simulink library "MBDS_Subsystems"  (R2018b)
settings: Solver=ode45  StartTime=0.0  StopTime=10.0  RelTol=1e-3
undefined symbols (not defined in the file or in its folder): nbo_False, nbo_True
libraries: KIBES_Signal x1438, MBDS_Modules x44, simulink x2
(part 11 of 15)

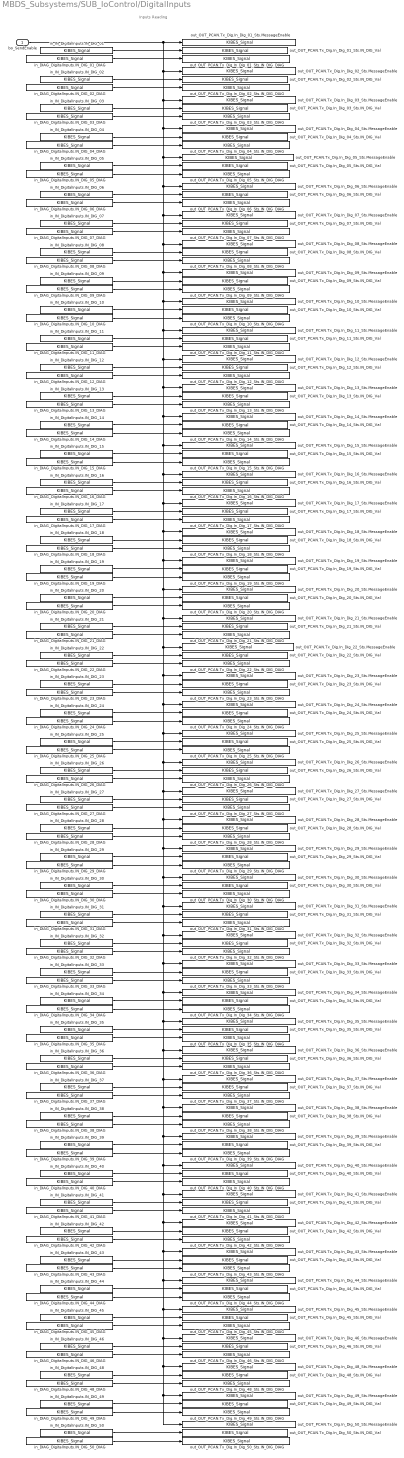
== system MBDS_Subsystems/SUB_IoControl/DigitalInputs ==
  note: Inputs Reading
  bo_SendEnable : Inport
  in_DIAG_DigitalInputs.IN_DIG_01_DIAG : KIBES_Signal/KIBES_Signal  MBDS_LibraryBlock=on  DatabaseKey=5  SignalName=DIAG_DigitalInputs.IN_DIG_01_DIAG  SymbolName=DIAG_DigitalInputs_IN_DIG_01_DIAG_000005  DataType=uint16  Init=1  Slope=1  Bias=0  DataSize=1  fpDataType=uint16  BlockIOType=Inport  DeviceType=0
  in_DIAG_DigitalInputs.IN_DIG_02_DIAG : KIBES_Signal/KIBES_Signal  MBDS_LibraryBlock=on  DatabaseKey=36  SignalName=DIAG_DigitalInputs.IN_DIG_02_DIAG  SymbolName=DIAG_DigitalInputs_IN_DIG_02_DIAG_000036  DataType=uint16  Init=1  Slope=1  Bias=0  DataSize=1  fpDataType=uint16  BlockIOType=Inport  DeviceType=0
  in_DIAG_DigitalInputs.IN_DIG_03_DIAG : KIBES_Signal/KIBES_Signal  MBDS_LibraryBlock=on  DatabaseKey=38  SignalName=DIAG_DigitalInputs.IN_DIG_03_DIAG  SymbolName=DIAG_DigitalInputs_IN_DIG_03_DIAG_000038  DataType=uint16  Init=1  Slope=1  Bias=0  DataSize=1  fpDataType=uint16  BlockIOType=Inport  DeviceType=0
  in_DIAG_DigitalInputs.IN_DIG_04_DIAG : KIBES_Signal/KIBES_Signal  MBDS_LibraryBlock=on  DatabaseKey=40  SignalName=DIAG_DigitalInputs.IN_DIG_04_DIAG  SymbolName=DIAG_DigitalInputs_IN_DIG_04_DIAG_000040  DataType=uint16  Init=1  Slope=1  Bias=0  DataSize=1  fpDataType=uint16  BlockIOType=Inport  DeviceType=0
  in_DIAG_DigitalInputs.IN_DIG_05_DIAG : KIBES_Signal/KIBES_Signal  MBDS_LibraryBlock=on  DatabaseKey=88  SignalName=DIAG_DigitalInputs.IN_DIG_05_DIAG  SymbolName=DIAG_DigitalInputs_IN_DIG_05_DIAG_000088  DataType=uint16  Init=1  Slope=1  Bias=0  DataSize=1  fpDataType=uint16  BlockIOType=Inport  DeviceType=0
  in_DIAG_DigitalInputs.IN_DIG_06_DIAG : KIBES_Signal/KIBES_Signal  MBDS_LibraryBlock=on  DatabaseKey=93  SignalName=DIAG_DigitalInputs.IN_DIG_06_DIAG  SymbolName=DIAG_DigitalInputs_IN_DIG_06_DIAG_000093  DataType=uint16  Init=1  Slope=1  Bias=0  DataSize=1  fpDataType=uint16  BlockIOType=Inport  DeviceType=0
  in_DIAG_DigitalInputs.IN_DIG_07_DIAG : KIBES_Signal/KIBES_Signal  MBDS_LibraryBlock=on  DatabaseKey=89  SignalName=DIAG_DigitalInputs.IN_DIG_07_DIAG  SymbolName=DIAG_DigitalInputs_IN_DIG_07_DIAG_000089  DataType=uint16  Init=1  Slope=1  Bias=0  DataSize=1  fpDataType=uint16  BlockIOType=Inport  DeviceType=0
  in_DIAG_DigitalInputs.IN_DIG_08_DIAG : KIBES_Signal/KIBES_Signal  MBDS_LibraryBlock=on  DatabaseKey=90  SignalName=DIAG_DigitalInputs.IN_DIG_08_DIAG  SymbolName=DIAG_DigitalInputs_IN_DIG_08_DIAG_000090  DataType=uint16  Init=1  Slope=1  Bias=0  DataSize=1  fpDataType=uint16  BlockIOType=Inport  DeviceType=0
  in_DIAG_DigitalInputs.IN_DIG_09_DIAG : KIBES_Signal/KIBES_Signal  MBDS_LibraryBlock=on  DatabaseKey=95  SignalName=DIAG_DigitalInputs.IN_DIG_09_DIAG  SymbolName=DIAG_DigitalInputs_IN_DIG_09_DIAG_000095  DataType=uint16  Init=1  Slope=1  Bias=0  DataSize=1  fpDataType=uint16  BlockIOType=Inport  DeviceType=0
  in_DIAG_DigitalInputs.IN_DIG_10_DIAG : KIBES_Signal/KIBES_Signal  MBDS_LibraryBlock=on  DatabaseKey=97  SignalName=DIAG_DigitalInputs.IN_DIG_10_DIAG  SymbolName=DIAG_DigitalInputs_IN_DIG_10_DIAG_000097  DataType=uint16  Init=1  Slope=1  Bias=0  DataSize=1  fpDataType=uint16  BlockIOType=Inport  DeviceType=0
  in_DIAG_DigitalInputs.IN_DIG_11_DIAG : KIBES_Signal/KIBES_Signal  MBDS_LibraryBlock=on  DatabaseKey=99  SignalName=DIAG_DigitalInputs.IN_DIG_11_DIAG  SymbolName=DIAG_DigitalInputs_IN_DIG_11_DIAG_000099  DataType=uint16  Init=1  Slope=1  Bias=0  DataSize=1  fpDataType=uint16  BlockIOType=Inport  DeviceType=0
  in_DIAG_DigitalInputs.IN_DIG_12_DIAG : KIBES_Signal/KIBES_Signal  MBDS_LibraryBlock=on  DatabaseKey=101  SignalName=DIAG_DigitalInputs.IN_DIG_12_DIAG  SymbolName=DIAG_DigitalInputs_IN_DIG_12_DIAG_000101  DataType=uint16  Init=1  Slope=1  Bias=0  DataSize=1  fpDataType=uint16  BlockIOType=Inport  DeviceType=0
  in_DIAG_DigitalInputs.IN_DIG_13_DIAG : KIBES_Signal/KIBES_Signal  MBDS_LibraryBlock=on  DatabaseKey=9  SignalName=DIAG_DigitalInputs.IN_DIG_13_DIAG  SymbolName=DIAG_DigitalInputs_IN_DIG_13_DIAG_000009  DataType=uint16  Init=1  Slope=1  Bias=0  DataSize=1  fpDataType=uint16  BlockIOType=Inport  DeviceType=0
  in_DIAG_DigitalInputs.IN_DIG_14_DIAG : KIBES_Signal/KIBES_Signal  MBDS_LibraryBlock=on  DatabaseKey=11  SignalName=DIAG_DigitalInputs.IN_DIG_14_DIAG  SymbolName=DIAG_DigitalInputs_IN_DIG_14_DIAG_000011  DataType=uint16  Init=1  Slope=1  Bias=0  DataSize=1  fpDataType=uint16  BlockIOType=Inport  DeviceType=0
  in_DIAG_DigitalInputs.IN_DIG_15_DIAG : KIBES_Signal/KIBES_Signal  MBDS_LibraryBlock=on  DatabaseKey=13  SignalName=DIAG_DigitalInputs.IN_DIG_15_DIAG  SymbolName=DIAG_DigitalInputs_IN_DIG_15_DIAG_000013  DataType=uint16  Init=1  Slope=1  Bias=0  DataSize=1  fpDataType=uint16  BlockIOType=Inport  DeviceType=0
  in_DIAG_DigitalInputs.IN_DIG_16_DIAG : KIBES_Signal/KIBES_Signal  MBDS_LibraryBlock=on  DatabaseKey=15  SignalName=DIAG_DigitalInputs.IN_DIG_16_DIAG  SymbolName=DIAG_DigitalInputs_IN_DIG_16_DIAG_000015  DataType=uint16  Init=1  Slope=1  Bias=0  DataSize=1  fpDataType=uint16  BlockIOType=Inport  DeviceType=0
  in_DIAG_DigitalInputs.IN_DIG_17_DIAG : KIBES_Signal/KIBES_Signal  MBDS_LibraryBlock=on  DatabaseKey=17  SignalName=DIAG_DigitalInputs.IN_DIG_17_DIAG  SymbolName=DIAG_DigitalInputs_IN_DIG_17_DIAG_000017  DataType=uint16  Init=1  Slope=1  Bias=0  DataSize=1  fpDataType=uint16  BlockIOType=Inport  DeviceType=0
  in_DIAG_DigitalInputs.IN_DIG_18_DIAG : KIBES_Signal/KIBES_Signal  MBDS_LibraryBlock=on  DatabaseKey=19  SignalName=DIAG_DigitalInputs.IN_DIG_18_DIAG  SymbolName=DIAG_DigitalInputs_IN_DIG_18_DIAG_000019  DataType=uint16  Init=1  Slope=1  Bias=0  DataSize=1  fpDataType=uint16  BlockIOType=Inport  DeviceType=0
  in_DIAG_DigitalInputs.IN_DIG_19_DIAG : KIBES_Signal/KIBES_Signal  MBDS_LibraryBlock=on  DatabaseKey=21  SignalName=DIAG_DigitalInputs.IN_DIG_19_DIAG  SymbolName=DIAG_DigitalInputs_IN_DIG_19_DIAG_000021  DataType=uint16  Init=1  Slope=1  Bias=0  DataSize=1  fpDataType=uint16  BlockIOType=Inport  DeviceType=0
  in_DIAG_DigitalInputs.IN_DIG_20_DIAG : KIBES_Signal/KIBES_Signal  MBDS_LibraryBlock=on  DatabaseKey=23  SignalName=DIAG_DigitalInputs.IN_DIG_20_DIAG  SymbolName=DIAG_DigitalInputs_IN_DIG_20_DIAG_000023  DataType=uint16  Init=1  Slope=1  Bias=0  DataSize=1  fpDataType=uint16  BlockIOType=Inport  DeviceType=0
  in_DIAG_DigitalInputs.IN_DIG_21_DIAG : KIBES_Signal/KIBES_Signal  MBDS_LibraryBlock=on  DatabaseKey=25  SignalName=DIAG_DigitalInputs.IN_DIG_21_DIAG  SymbolName=DIAG_DigitalInputs_IN_DIG_21_DIAG_000025  DataType=uint16  Init=1  Slope=1  Bias=0  DataSize=1  fpDataType=uint16  BlockIOType=Inport  DeviceType=0
  in_DIAG_DigitalInputs.IN_DIG_22_DIAG : KIBES_Signal/KIBES_Signal  MBDS_LibraryBlock=on  DatabaseKey=27  SignalName=DIAG_DigitalInputs.IN_DIG_22_DIAG  SymbolName=DIAG_DigitalInputs_IN_DIG_22_DIAG_000027  DataType=uint16  Init=1  Slope=1  Bias=0  DataSize=1  fpDataType=uint16  BlockIOType=Inport  DeviceType=0
  in_DIAG_DigitalInputs.IN_DIG_23_DIAG : KIBES_Signal/KIBES_Signal  MBDS_LibraryBlock=on  DatabaseKey=29  SignalName=DIAG_DigitalInputs.IN_DIG_23_DIAG  SymbolName=DIAG_DigitalInputs_IN_DIG_23_DIAG_000029  DataType=uint16  Init=1  Slope=1  Bias=0  DataSize=1  fpDataType=uint16  BlockIOType=Inport  DeviceType=0
  in_DIAG_DigitalInputs.IN_DIG_24_DIAG : KIBES_Signal/KIBES_Signal  MBDS_LibraryBlock=on  DatabaseKey=31  SignalName=DIAG_DigitalInputs.IN_DIG_24_DIAG  SymbolName=DIAG_DigitalInputs_IN_DIG_24_DIAG_000031  DataType=uint16  Init=1  Slope=1  Bias=0  DataSize=1  fpDataType=uint16  BlockIOType=Inport  DeviceType=0
  in_DIAG_DigitalInputs.IN_DIG_25_DIAG : KIBES_Signal/KIBES_Signal  MBDS_LibraryBlock=on  DatabaseKey=33  SignalName=DIAG_DigitalInputs.IN_DIG_25_DIAG  SymbolName=DIAG_DigitalInputs_IN_DIG_25_DIAG_000033  DataType=uint16  Init=1  Slope=1  Bias=0  DataSize=1  fpDataType=uint16  BlockIOType=Inport  DeviceType=0
  in_DIAG_DigitalInputs.IN_DIG_26_DIAG : KIBES_Signal/KIBES_Signal  MBDS_LibraryBlock=on  DatabaseKey=41  SignalName=DIAG_DigitalInputs.IN_DIG_26_DIAG  SymbolName=DIAG_DigitalInputs_IN_DIG_26_DIAG_000041  DataType=uint16  Init=1  Slope=1  Bias=0  DataSize=1  fpDataType=uint16  BlockIOType=Inport  DeviceType=0
  in_DIAG_DigitalInputs.IN_DIG_27_DIAG : KIBES_Signal/KIBES_Signal  MBDS_LibraryBlock=on  DatabaseKey=43  SignalName=DIAG_DigitalInputs.IN_DIG_27_DIAG  SymbolName=DIAG_DigitalInputs_IN_DIG_27_DIAG_000043  DataType=uint16  Init=1  Slope=1  Bias=0  DataSize=1  fpDataType=uint16  BlockIOType=Inport  DeviceType=0
  in_DIAG_DigitalInputs.IN_DIG_28_DIAG : KIBES_Signal/KIBES_Signal  MBDS_LibraryBlock=on  DatabaseKey=45  SignalName=DIAG_DigitalInputs.IN_DIG_28_DIAG  SymbolName=DIAG_DigitalInputs_IN_DIG_28_DIAG_000045  DataType=uint16  Init=1  Slope=1  Bias=0  DataSize=1  fpDataType=uint16  BlockIOType=Inport  DeviceType=0
  in_DIAG_DigitalInputs.IN_DIG_29_DIAG : KIBES_Signal/KIBES_Signal  MBDS_LibraryBlock=on  DatabaseKey=47  SignalName=DIAG_DigitalInputs.IN_DIG_29_DIAG  SymbolName=DIAG_DigitalInputs_IN_DIG_29_DIAG_000047  DataType=uint16  Init=1  Slope=1  Bias=0  DataSize=1  fpDataType=uint16  BlockIOType=Inport  DeviceType=0
  in_DIAG_DigitalInputs.IN_DIG_30_DIAG : KIBES_Signal/KIBES_Signal  MBDS_LibraryBlock=on  DatabaseKey=49  SignalName=DIAG_DigitalInputs.IN_DIG_30_DIAG  SymbolName=DIAG_DigitalInputs_IN_DIG_30_DIAG_000049  DataType=uint16  Init=1  Slope=1  Bias=0  DataSize=1  fpDataType=uint16  BlockIOType=Inport  DeviceType=0
  in_DIAG_DigitalInputs.IN_DIG_31_DIAG : KIBES_Signal/KIBES_Signal  MBDS_LibraryBlock=on  DatabaseKey=51  SignalName=DIAG_DigitalInputs.IN_DIG_31_DIAG  SymbolName=DIAG_DigitalInputs_IN_DIG_31_DIAG_000051  DataType=uint16  Init=1  Slope=1  Bias=0  DataSize=1  fpDataType=uint16  BlockIOType=Inport  DeviceType=0
  in_DIAG_DigitalInputs.IN_DIG_32_DIAG : KIBES_Signal/KIBES_Signal  MBDS_LibraryBlock=on  DatabaseKey=53  SignalName=DIAG_DigitalInputs.IN_DIG_32_DIAG  SymbolName=DIAG_DigitalInputs_IN_DIG_32_DIAG_000053  DataType=uint16  Init=1  Slope=1  Bias=0  DataSize=1  fpDataType=uint16  BlockIOType=Inport  DeviceType=0
  in_DIAG_DigitalInputs.IN_DIG_33_DIAG : KIBES_Signal/KIBES_Signal  MBDS_LibraryBlock=on  DatabaseKey=55  SignalName=DIAG_DigitalInputs.IN_DIG_33_DIAG  SymbolName=DIAG_DigitalInputs_IN_DIG_33_DIAG_000055  DataType=uint16  Init=1  Slope=1  Bias=0  DataSize=1  fpDataType=uint16  BlockIOType=Inport  DeviceType=0
  in_DIAG_DigitalInputs.IN_DIG_34_DIAG : KIBES_Signal/KIBES_Signal  MBDS_LibraryBlock=on  DatabaseKey=57  SignalName=DIAG_DigitalInputs.IN_DIG_34_DIAG  SymbolName=DIAG_DigitalInputs_IN_DIG_34_DIAG_000057  DataType=uint16  Init=1  Slope=1  Bias=0  DataSize=1  fpDataType=uint16  BlockIOType=Inport  DeviceType=0
  in_DIAG_DigitalInputs.IN_DIG_35_DIAG : KIBES_Signal/KIBES_Signal  MBDS_LibraryBlock=on  DatabaseKey=59  SignalName=DIAG_DigitalInputs.IN_DIG_35_DIAG  SymbolName=DIAG_DigitalInputs_IN_DIG_35_DIAG_000059  DataType=uint16  Init=1  Slope=1  Bias=0  DataSize=1  fpDataType=uint16  BlockIOType=Inport  DeviceType=0
  in_DIAG_DigitalInputs.IN_DIG_36_DIAG : KIBES_Signal/KIBES_Signal  MBDS_LibraryBlock=on  DatabaseKey=61  SignalName=DIAG_DigitalInputs.IN_DIG_36_DIAG  SymbolName=DIAG_DigitalInputs_IN_DIG_36_DIAG_000061  DataType=uint16  Init=1  Slope=1  Bias=0  DataSize=1  fpDataType=uint16  BlockIOType=Inport  DeviceType=0
  in_DIAG_DigitalInputs.IN_DIG_37_DIAG : KIBES_Signal/KIBES_Signal  MBDS_LibraryBlock=on  DatabaseKey=63  SignalName=DIAG_DigitalInputs.IN_DIG_37_DIAG  SymbolName=DIAG_DigitalInputs_IN_DIG_37_DIAG_000063  DataType=uint16  Init=1  Slope=1  Bias=0  DataSize=1  fpDataType=uint16  BlockIOType=Inport  DeviceType=0
  in_DIAG_DigitalInputs.IN_DIG_38_DIAG : KIBES_Signal/KIBES_Signal  MBDS_LibraryBlock=on  DatabaseKey=65  SignalName=DIAG_DigitalInputs.IN_DIG_38_DIAG  SymbolName=DIAG_DigitalInputs_IN_DIG_38_DIAG_000065  DataType=uint16  Init=1  Slope=1  Bias=0  DataSize=1  fpDataType=uint16  BlockIOType=Inport  DeviceType=0
  in_DIAG_DigitalInputs.IN_DIG_39_DIAG : KIBES_Signal/KIBES_Signal  MBDS_LibraryBlock=on  DatabaseKey=67  SignalName=DIAG_DigitalInputs.IN_DIG_39_DIAG  SymbolName=DIAG_DigitalInputs_IN_DIG_39_DIAG_000067  DataType=uint16  Init=1  Slope=1  Bias=0  DataSize=1  fpDataType=uint16  BlockIOType=Inport  DeviceType=0
  in_DIAG_DigitalInputs.IN_DIG_40_DIAG : KIBES_Signal/KIBES_Signal  MBDS_LibraryBlock=on  DatabaseKey=69  SignalName=DIAG_DigitalInputs.IN_DIG_40_DIAG  SymbolName=DIAG_DigitalInputs_IN_DIG_40_DIAG_000069  DataType=uint16  Init=1  Slope=1  Bias=0  DataSize=1  fpDataType=uint16  BlockIOType=Inport  DeviceType=0
  in_DIAG_DigitalInputs.IN_DIG_41_DIAG : KIBES_Signal/KIBES_Signal  MBDS_LibraryBlock=on  DatabaseKey=71  SignalName=DIAG_DigitalInputs.IN_DIG_41_DIAG  SymbolName=DIAG_DigitalInputs_IN_DIG_41_DIAG_000071  DataType=uint16  Init=1  Slope=1  Bias=0  DataSize=1  fpDataType=uint16  BlockIOType=Inport  DeviceType=0
  in_DIAG_DigitalInputs.IN_DIG_42_DIAG : KIBES_Signal/KIBES_Signal  MBDS_LibraryBlock=on  DatabaseKey=73  SignalName=DIAG_DigitalInputs.IN_DIG_42_DIAG  SymbolName=DIAG_DigitalInputs_IN_DIG_42_DIAG_000073  DataType=uint16  Init=1  Slope=1  Bias=0  DataSize=1  fpDataType=uint16  BlockIOType=Inport  DeviceType=0
  in_DIAG_DigitalInputs.IN_DIG_43_DIAG : KIBES_Signal/KIBES_Signal  MBDS_LibraryBlock=on  DatabaseKey=75  SignalName=DIAG_DigitalInputs.IN_DIG_43_DIAG  SymbolName=DIAG_DigitalInputs_IN_DIG_43_DIAG_000075  DataType=uint16  Init=1  Slope=1  Bias=0  DataSize=1  fpDataType=uint16  BlockIOType=Inport  DeviceType=0
  in_DIAG_DigitalInputs.IN_DIG_44_DIAG : KIBES_Signal/KIBES_Signal  MBDS_LibraryBlock=on  DatabaseKey=77  SignalName=DIAG_DigitalInputs.IN_DIG_44_DIAG  SymbolName=DIAG_DigitalInputs_IN_DIG_44_DIAG_000077  DataType=uint16  Init=1  Slope=1  Bias=0  DataSize=1  fpDataType=uint16  BlockIOType=Inport  DeviceType=0
  in_DIAG_DigitalInputs.IN_DIG_45_DIAG : KIBES_Signal/KIBES_Signal  MBDS_LibraryBlock=on  DatabaseKey=79  SignalName=DIAG_DigitalInputs.IN_DIG_45_DIAG  SymbolName=DIAG_DigitalInputs_IN_DIG_45_DIAG_000079  DataType=uint16  Init=1  Slope=1  Bias=0  DataSize=1  fpDataType=uint16  BlockIOType=Inport  DeviceType=0
  in_DIAG_DigitalInputs.IN_DIG_46_DIAG : KIBES_Signal/KIBES_Signal  MBDS_LibraryBlock=on  DatabaseKey=81  SignalName=DIAG_DigitalInputs.IN_DIG_46_DIAG  SymbolName=DIAG_DigitalInputs_IN_DIG_46_DIAG_000081  DataType=uint16  Init=1  Slope=1  Bias=0  DataSize=1  fpDataType=uint16  BlockIOType=Inport  DeviceType=0
  in_DIAG_DigitalInputs.IN_DIG_48_DIAG : KIBES_Signal/KIBES_Signal  MBDS_LibraryBlock=on  DatabaseKey=83  SignalName=DIAG_DigitalInputs.IN_DIG_48_DIAG  SymbolName=DIAG_DigitalInputs_IN_DIG_48_DIAG_000083  DataType=uint16  Init=1  Slope=1  Bias=0  DataSize=1  fpDataType=uint16  BlockIOType=Inport  DeviceType=0
  in_DIAG_DigitalInputs.IN_DIG_49_DIAG : KIBES_Signal/KIBES_Signal  MBDS_LibraryBlock=on  DatabaseKey=85  SignalName=DIAG_DigitalInputs.IN_DIG_49_DIAG  SymbolName=DIAG_DigitalInputs_IN_DIG_49_DIAG_000085  DataType=uint16  Init=1  Slope=1  Bias=0  DataSize=1  fpDataType=uint16  BlockIOType=Inport  DeviceType=0
  in_DIAG_DigitalInputs.IN_DIG_50_DIAG : KIBES_Signal/KIBES_Signal  MBDS_LibraryBlock=on  DatabaseKey=91  SignalName=DIAG_DigitalInputs.IN_DIG_50_DIAG  SymbolName=DIAG_DigitalInputs_IN_DIG_50_DIAG_000091  DataType=uint16  Init=1  Slope=1  Bias=0  DataSize=1  fpDataType=uint16  BlockIOType=Inport  DeviceType=0
  in_IN_DigitalInputs.IN_DIG_01 : KIBES_Signal/KIBES_Signal  MBDS_LibraryBlock=on  DatabaseKey=4  SignalName=IN_DigitalInputs.IN_DIG_01  SymbolName=IN_DigitalInputs_IN_DIG_01_000004  DataType=boolean  Init=0  Slope=1  Bias=0  DataSize=1  fpDataType=boolean  BlockIOType=Inport  DeviceType=0
  in_IN_DigitalInputs.IN_DIG_02 : KIBES_Signal/KIBES_Signal  MBDS_LibraryBlock=on  DatabaseKey=35  SignalName=IN_DigitalInputs.IN_DIG_02  SymbolName=IN_DigitalInputs_IN_DIG_02_000035  DataType=boolean  Init=0  Slope=1  Bias=0  DataSize=1  fpDataType=boolean  BlockIOType=Inport  DeviceType=0
  in_IN_DigitalInputs.IN_DIG_03 : KIBES_Signal/KIBES_Signal  MBDS_LibraryBlock=on  DatabaseKey=37  SignalName=IN_DigitalInputs.IN_DIG_03  SymbolName=IN_DigitalInputs_IN_DIG_03_000037  DataType=boolean  Init=0  Slope=1  Bias=0  DataSize=1  fpDataType=boolean  BlockIOType=Inport  DeviceType=0
  in_IN_DigitalInputs.IN_DIG_04 : KIBES_Signal/KIBES_Signal  MBDS_LibraryBlock=on  DatabaseKey=39  SignalName=IN_DigitalInputs.IN_DIG_04  SymbolName=IN_DigitalInputs_IN_DIG_04_000039  DataType=boolean  Init=0  Slope=1  Bias=0  DataSize=1  fpDataType=boolean  BlockIOType=Inport  DeviceType=0
  in_IN_DigitalInputs.IN_DIG_05 : KIBES_Signal/KIBES_Signal  MBDS_LibraryBlock=on  DatabaseKey=87  SignalName=IN_DigitalInputs.IN_DIG_05  SymbolName=IN_DigitalInputs_IN_DIG_05_000087  DataType=boolean  Init=0  Slope=1  Bias=0  DataSize=1  fpDataType=boolean  BlockIOType=Inport  DeviceType=0
  in_IN_DigitalInputs.IN_DIG_06 : KIBES_Signal/KIBES_Signal  MBDS_LibraryBlock=on  DatabaseKey=92  SignalName=IN_DigitalInputs.IN_DIG_06  SymbolName=IN_DigitalInputs_IN_DIG_06_000092  DataType=boolean  Init=0  Slope=1  Bias=0  DataSize=1  fpDataType=boolean  BlockIOType=Inport  DeviceType=0
  in_IN_DigitalInputs.IN_DIG_07 : KIBES_Signal/KIBES_Signal  MBDS_LibraryBlock=on  DatabaseKey=6  SignalName=IN_DigitalInputs.IN_DIG_07  SymbolName=IN_DigitalInputs_IN_DIG_07_000006  DataType=boolean  Init=0  Slope=1  Bias=0  DataSize=1  fpDataType=boolean  BlockIOType=Inport  DeviceType=0
  in_IN_DigitalInputs.IN_DIG_08 : KIBES_Signal/KIBES_Signal  MBDS_LibraryBlock=on  DatabaseKey=7  SignalName=IN_DigitalInputs.IN_DIG_08  SymbolName=IN_DigitalInputs_IN_DIG_08_000007  DataType=boolean  Init=0  Slope=1  Bias=0  DataSize=1  fpDataType=boolean  BlockIOType=Inport  DeviceType=0
  in_IN_DigitalInputs.IN_DIG_09 : KIBES_Signal/KIBES_Signal  MBDS_LibraryBlock=on  DatabaseKey=94  SignalName=IN_DigitalInputs.IN_DIG_09  SymbolName=IN_DigitalInputs_IN_DIG_09_000094  DataType=boolean  Init=0  Slope=1  Bias=0  DataSize=1  fpDataType=boolean  BlockIOType=Inport  DeviceType=0
  in_IN_DigitalInputs.IN_DIG_10 : KIBES_Signal/KIBES_Signal  MBDS_LibraryBlock=on  DatabaseKey=96  SignalName=IN_DigitalInputs.IN_DIG_10  SymbolName=IN_DigitalInputs_IN_DIG_10_000096  DataType=boolean  Init=0  Slope=1  Bias=0  DataSize=1  fpDataType=boolean  BlockIOType=Inport  DeviceType=0
  in_IN_DigitalInputs.IN_DIG_11 : KIBES_Signal/KIBES_Signal  MBDS_LibraryBlock=on  DatabaseKey=98  SignalName=IN_DigitalInputs.IN_DIG_11  SymbolName=IN_DigitalInputs_IN_DIG_11_000098  DataType=boolean  Init=0  Slope=1  Bias=0  DataSize=1  fpDataType=boolean  BlockIOType=Inport  DeviceType=0
  in_IN_DigitalInputs.IN_DIG_12 : KIBES_Signal/KIBES_Signal  MBDS_LibraryBlock=on  DatabaseKey=100  SignalName=IN_DigitalInputs.IN_DIG_12  SymbolName=IN_DigitalInputs_IN_DIG_12_000100  DataType=boolean  Init=0  Slope=1  Bias=0  DataSize=1  fpDataType=boolean  BlockIOType=Inport  DeviceType=0
  in_IN_DigitalInputs.IN_DIG_13 : KIBES_Signal/KIBES_Signal  MBDS_LibraryBlock=on  DatabaseKey=8  SignalName=IN_DigitalInputs.IN_DIG_13  SymbolName=IN_DigitalInputs_IN_DIG_13_000008  DataType=boolean  Init=0  Slope=1  Bias=0  DataSize=1  fpDataType=boolean  BlockIOType=Inport  DeviceType=0
  in_IN_DigitalInputs.IN_DIG_14 : KIBES_Signal/KIBES_Signal  MBDS_LibraryBlock=on  DatabaseKey=10  SignalName=IN_DigitalInputs.IN_DIG_14  SymbolName=IN_DigitalInputs_IN_DIG_14_000010  DataType=boolean  Init=0  Slope=1  Bias=0  DataSize=1  fpDataType=boolean  BlockIOType=Inport  DeviceType=0
  in_IN_DigitalInputs.IN_DIG_15 : KIBES_Signal/KIBES_Signal  MBDS_LibraryBlock=on  DatabaseKey=12  SignalName=IN_DigitalInputs.IN_DIG_15  SymbolName=IN_DigitalInputs_IN_DIG_15_000012  DataType=boolean  Init=0  Slope=1  Bias=0  DataSize=1  fpDataType=boolean  BlockIOType=Inport  DeviceType=0
  in_IN_DigitalInputs.IN_DIG_16 : KIBES_Signal/KIBES_Signal  MBDS_LibraryBlock=on  DatabaseKey=14  SignalName=IN_DigitalInputs.IN_DIG_16  SymbolName=IN_DigitalInputs_IN_DIG_16_000014  DataType=boolean  Init=0  Slope=1  Bias=0  DataSize=1  fpDataType=boolean  BlockIOType=Inport  DeviceType=0
  in_IN_DigitalInputs.IN_DIG_17 : KIBES_Signal/KIBES_Signal  MBDS_LibraryBlock=on  DatabaseKey=16  SignalName=IN_DigitalInputs.IN_DIG_17  SymbolName=IN_DigitalInputs_IN_DIG_17_000016  DataType=boolean  Init=0  Slope=1  Bias=0  DataSize=1  fpDataType=boolean  BlockIOType=Inport  DeviceType=0
  in_IN_DigitalInputs.IN_DIG_18 : KIBES_Signal/KIBES_Signal  MBDS_LibraryBlock=on  DatabaseKey=18  SignalName=IN_DigitalInputs.IN_DIG_18  SymbolName=IN_DigitalInputs_IN_DIG_18_000018  DataType=boolean  Init=0  Slope=1  Bias=0  DataSize=1  fpDataType=boolean  BlockIOType=Inport  DeviceType=0
  in_IN_DigitalInputs.IN_DIG_19 : KIBES_Signal/KIBES_Signal  MBDS_LibraryBlock=on  DatabaseKey=20  SignalName=IN_DigitalInputs.IN_DIG_19  SymbolName=IN_DigitalInputs_IN_DIG_19_000020  DataType=boolean  Init=0  Slope=1  Bias=0  DataSize=1  fpDataType=boolean  BlockIOType=Inport  DeviceType=0
  in_IN_DigitalInputs.IN_DIG_20 : KIBES_Signal/KIBES_Signal  MBDS_LibraryBlock=on  DatabaseKey=22  SignalName=IN_DigitalInputs.IN_DIG_20  SymbolName=IN_DigitalInputs_IN_DIG_20_000022  DataType=boolean  Init=0  Slope=1  Bias=0  DataSize=1  fpDataType=boolean  BlockIOType=Inport  DeviceType=0
  in_IN_DigitalInputs.IN_DIG_21 : KIBES_Signal/KIBES_Signal  MBDS_LibraryBlock=on  DatabaseKey=24  SignalName=IN_DigitalInputs.IN_DIG_21  SymbolName=IN_DigitalInputs_IN_DIG_21_000024  DataType=boolean  Init=0  Slope=1  Bias=0  DataSize=1  fpDataType=boolean  BlockIOType=Inport  DeviceType=0
  in_IN_DigitalInputs.IN_DIG_22 : KIBES_Signal/KIBES_Signal  MBDS_LibraryBlock=on  DatabaseKey=26  SignalName=IN_DigitalInputs.IN_DIG_22  SymbolName=IN_DigitalInputs_IN_DIG_22_000026  DataType=boolean  Init=0  Slope=1  Bias=0  DataSize=1  fpDataType=boolean  BlockIOType=Inport  DeviceType=0
  in_IN_DigitalInputs.IN_DIG_23 : KIBES_Signal/KIBES_Signal  MBDS_LibraryBlock=on  DatabaseKey=28  SignalName=IN_DigitalInputs.IN_DIG_23  SymbolName=IN_DigitalInputs_IN_DIG_23_000028  DataType=boolean  Init=0  Slope=1  Bias=0  DataSize=1  fpDataType=boolean  BlockIOType=Inport  DeviceType=0
  in_IN_DigitalInputs.IN_DIG_24 : KIBES_Signal/KIBES_Signal  MBDS_LibraryBlock=on  DatabaseKey=30  SignalName=IN_DigitalInputs.IN_DIG_24  SymbolName=IN_DigitalInputs_IN_DIG_24_000030  DataType=boolean  Init=0  Slope=1  Bias=0  DataSize=1  fpDataType=boolean  BlockIOType=Inport  DeviceType=0
  in_IN_DigitalInputs.IN_DIG_25 : KIBES_Signal/KIBES_Signal  MBDS_LibraryBlock=on  DatabaseKey=32  SignalName=IN_DigitalInputs.IN_DIG_25  SymbolName=IN_DigitalInputs_IN_DIG_25_000032  DataType=boolean  Init=0  Slope=1  Bias=0  DataSize=1  fpDataType=boolean  BlockIOType=Inport  DeviceType=0
  in_IN_DigitalInputs.IN_DIG_26 : KIBES_Signal/KIBES_Signal  MBDS_LibraryBlock=on  DatabaseKey=34  SignalName=IN_DigitalInputs.IN_DIG_26  SymbolName=IN_DigitalInputs_IN_DIG_26_000034  DataType=boolean  Init=0  Slope=1  Bias=0  DataSize=1  fpDataType=boolean  BlockIOType=Inport  DeviceType=0
  in_IN_DigitalInputs.IN_DIG_27 : KIBES_Signal/KIBES_Signal  MBDS_LibraryBlock=on  DatabaseKey=42  SignalName=IN_DigitalInputs.IN_DIG_27  SymbolName=IN_DigitalInputs_IN_DIG_27_000042  DataType=boolean  Init=0  Slope=1  Bias=0  DataSize=1  fpDataType=boolean  BlockIOType=Inport  DeviceType=0
  in_IN_DigitalInputs.IN_DIG_28 : KIBES_Signal/KIBES_Signal  MBDS_LibraryBlock=on  DatabaseKey=44  SignalName=IN_DigitalInputs.IN_DIG_28  SymbolName=IN_DigitalInputs_IN_DIG_28_000044  DataType=boolean  Init=0  Slope=1  Bias=0  DataSize=1  fpDataType=boolean  BlockIOType=Inport  DeviceType=0
  in_IN_DigitalInputs.IN_DIG_29 : KIBES_Signal/KIBES_Signal  MBDS_LibraryBlock=on  DatabaseKey=46  SignalName=IN_DigitalInputs.IN_DIG_29  SymbolName=IN_DigitalInputs_IN_DIG_29_000046  DataType=boolean  Init=0  Slope=1  Bias=0  DataSize=1  fpDataType=boolean  BlockIOType=Inport  DeviceType=0
  in_IN_DigitalInputs.IN_DIG_30 : KIBES_Signal/KIBES_Signal  MBDS_LibraryBlock=on  DatabaseKey=48  SignalName=IN_DigitalInputs.IN_DIG_30  SymbolName=IN_DigitalInputs_IN_DIG_30_000048  DataType=boolean  Init=0  Slope=1  Bias=0  DataSize=1  fpDataType=boolean  BlockIOType=Inport  DeviceType=0
  in_IN_DigitalInputs.IN_DIG_31 : KIBES_Signal/KIBES_Signal  MBDS_LibraryBlock=on  DatabaseKey=50  SignalName=IN_DigitalInputs.IN_DIG_31  SymbolName=IN_DigitalInputs_IN_DIG_31_000050  DataType=boolean  Init=0  Slope=1  Bias=0  DataSize=1  fpDataType=boolean  BlockIOType=Inport  DeviceType=0
  in_IN_DigitalInputs.IN_DIG_32 : KIBES_Signal/KIBES_Signal  MBDS_LibraryBlock=on  DatabaseKey=52  SignalName=IN_DigitalInputs.IN_DIG_32  SymbolName=IN_DigitalInputs_IN_DIG_32_000052  DataType=boolean  Init=0  Slope=1  Bias=0  DataSize=1  fpDataType=boolean  BlockIOType=Inport  DeviceType=0
  in_IN_DigitalInputs.IN_DIG_33 : KIBES_Signal/KIBES_Signal  MBDS_LibraryBlock=on  DatabaseKey=54  SignalName=IN_DigitalInputs.IN_DIG_33  SymbolName=IN_DigitalInputs_IN_DIG_33_000054  DataType=boolean  Init=0  Slope=1  Bias=0  DataSize=1  fpDataType=boolean  BlockIOType=Inport  DeviceType=0
  in_IN_DigitalInputs.IN_DIG_34 : KIBES_Signal/KIBES_Signal  MBDS_LibraryBlock=on  DatabaseKey=56  SignalName=IN_DigitalInputs.IN_DIG_34  SymbolName=IN_DigitalInputs_IN_DIG_34_000056  DataType=boolean  Init=0  Slope=1  Bias=0  DataSize=1  fpDataType=boolean  BlockIOType=Inport  DeviceType=0
  in_IN_DigitalInputs.IN_DIG_35 : KIBES_Signal/KIBES_Signal  MBDS_LibraryBlock=on  DatabaseKey=58  SignalName=IN_DigitalInputs.IN_DIG_35  SymbolName=IN_DigitalInputs_IN_DIG_35_000058  DataType=boolean  Init=0  Slope=1  Bias=0  DataSize=1  fpDataType=boolean  BlockIOType=Inport  DeviceType=0
  in_IN_DigitalInputs.IN_DIG_36 : KIBES_Signal/KIBES_Signal  MBDS_LibraryBlock=on  DatabaseKey=60  SignalName=IN_DigitalInputs.IN_DIG_36  SymbolName=IN_DigitalInputs_IN_DIG_36_000060  DataType=boolean  Init=0  Slope=1  Bias=0  DataSize=1  fpDataType=boolean  BlockIOType=Inport  DeviceType=0
  in_IN_DigitalInputs.IN_DIG_37 : KIBES_Signal/KIBES_Signal  MBDS_LibraryBlock=on  DatabaseKey=62  SignalName=IN_DigitalInputs.IN_DIG_37  SymbolName=IN_DigitalInputs_IN_DIG_37_000062  DataType=boolean  Init=0  Slope=1  Bias=0  DataSize=1  fpDataType=boolean  BlockIOType=Inport  DeviceType=0
  in_IN_DigitalInputs.IN_DIG_38 : KIBES_Signal/KIBES_Signal  MBDS_LibraryBlock=on  DatabaseKey=64  SignalName=IN_DigitalInputs.IN_DIG_38  SymbolName=IN_DigitalInputs_IN_DIG_38_000064  DataType=boolean  Init=0  Slope=1  Bias=0  DataSize=1  fpDataType=boolean  BlockIOType=Inport  DeviceType=0
  in_IN_DigitalInputs.IN_DIG_39 : KIBES_Signal/KIBES_Signal  MBDS_LibraryBlock=on  DatabaseKey=66  SignalName=IN_DigitalInputs.IN_DIG_39  SymbolName=IN_DigitalInputs_IN_DIG_39_000066  DataType=boolean  Init=0  Slope=1  Bias=0  DataSize=1  fpDataType=boolean  BlockIOType=Inport  DeviceType=0
  in_IN_DigitalInputs.IN_DIG_40 : KIBES_Signal/KIBES_Signal  MBDS_LibraryBlock=on  DatabaseKey=68  SignalName=IN_DigitalInputs.IN_DIG_40  SymbolName=IN_DigitalInputs_IN_DIG_40_000068  DataType=boolean  Init=0  Slope=1  Bias=0  DataSize=1  fpDataType=boolean  BlockIOType=Inport  DeviceType=0
  in_IN_DigitalInputs.IN_DIG_41 : KIBES_Signal/KIBES_Signal  MBDS_LibraryBlock=on  DatabaseKey=70  SignalName=IN_DigitalInputs.IN_DIG_41  SymbolName=IN_DigitalInputs_IN_DIG_41_000070  DataType=boolean  Init=0  Slope=1  Bias=0  DataSize=1  fpDataType=boolean  BlockIOType=Inport  DeviceType=0
  in_IN_DigitalInputs.IN_DIG_42 : KIBES_Signal/KIBES_Signal  MBDS_LibraryBlock=on  DatabaseKey=72  SignalName=IN_DigitalInputs.IN_DIG_42  SymbolName=IN_DigitalInputs_IN_DIG_42_000072  DataType=boolean  Init=0  Slope=1  Bias=0  DataSize=1  fpDataType=boolean  BlockIOType=Inport  DeviceType=0
  in_IN_DigitalInputs.IN_DIG_43 : KIBES_Signal/KIBES_Signal  MBDS_LibraryBlock=on  DatabaseKey=74  SignalName=IN_DigitalInputs.IN_DIG_43  SymbolName=IN_DigitalInputs_IN_DIG_43_000074  DataType=boolean  Init=0  Slope=1  Bias=0  DataSize=1  fpDataType=boolean  BlockIOType=Inport  DeviceType=0
  in_IN_DigitalInputs.IN_DIG_44 : KIBES_Signal/KIBES_Signal  MBDS_LibraryBlock=on  DatabaseKey=76  SignalName=IN_DigitalInputs.IN_DIG_44  SymbolName=IN_DigitalInputs_IN_DIG_44_000076  DataType=boolean  Init=0  Slope=1  Bias=0  DataSize=1  fpDataType=boolean  BlockIOType=Inport  DeviceType=0
  in_IN_DigitalInputs.IN_DIG_45 : KIBES_Signal/KIBES_Signal  MBDS_LibraryBlock=on  DatabaseKey=78  SignalName=IN_DigitalInputs.IN_DIG_45  SymbolName=IN_DigitalInputs_IN_DIG_45_000078  DataType=boolean  Init=0  Slope=1  Bias=0  DataSize=1  fpDataType=boolean  BlockIOType=Inport  DeviceType=0
  in_IN_DigitalInputs.IN_DIG_46 : KIBES_Signal/KIBES_Signal  MBDS_LibraryBlock=on  DatabaseKey=80  SignalName=IN_DigitalInputs.IN_DIG_46  SymbolName=IN_DigitalInputs_IN_DIG_46_000080  DataType=boolean  Init=0  Slope=1  Bias=0  DataSize=1  fpDataType=boolean  BlockIOType=Inport  DeviceType=0
  in_IN_DigitalInputs.IN_DIG_48 : KIBES_Signal/KIBES_Signal  MBDS_LibraryBlock=on  DatabaseKey=82  SignalName=IN_DigitalInputs.IN_DIG_48  SymbolName=IN_DigitalInputs_IN_DIG_48_000082  DataType=boolean  Init=0  Slope=1  Bias=0  DataSize=1  fpDataType=boolean  BlockIOType=Inport  DeviceType=0
  in_IN_DigitalInputs.IN_DIG_49 : KIBES_Signal/KIBES_Signal  MBDS_LibraryBlock=on  DatabaseKey=84  SignalName=IN_DigitalInputs.IN_DIG_49  SymbolName=IN_DigitalInputs_IN_DIG_49_000084  DataType=boolean  Init=0  Slope=1  Bias=0  DataSize=1  fpDataType=boolean  BlockIOType=Inport  DeviceType=0
  in_IN_DigitalInputs.IN_DIG_50 : KIBES_Signal/KIBES_Signal  MBDS_LibraryBlock=on  DatabaseKey=86  SignalName=IN_DigitalInputs.IN_DIG_50  SymbolName=IN_DigitalInputs_IN_DIG_50_000086  DataType=boolean  Init=0  Slope=1  Bias=0  DataSize=1  fpDataType=boolean  BlockIOType=Inport  DeviceType=0
  out_OUT_PCAN.Tx_Dig.In_Dig_01_Sts.IN_DIG_DIAG : KIBES_Signal/KIBES_Signal  MBDS_LibraryBlock=on  DatabaseKey=1401  SignalName=OUT_PCAN.Tx_Dig.In_Dig_01_Sts.IN_DIG_DIAG  SymbolName=OUT_PCAN_Tx_Dig_In_Dig_01_Sts_IN_DIG_DIAG_001401  DataType=uint16  Init=0  Slope=1  Bias=0  DataSize=1  fpDataType=uint16  BlockIOType=Outport  DeviceType=0
  out_OUT_PCAN.Tx_Dig.In_Dig_01_Sts.IN_DIG_Val : KIBES_Signal/KIBES_Signal  MBDS_LibraryBlock=on  DatabaseKey=1402  SignalName=OUT_PCAN.Tx_Dig.In_Dig_01_Sts.IN_DIG_Val  SymbolName=OUT_PCAN_Tx_Dig_In_Dig_01_Sts_IN_DIG_Val_001402  DataType=boolean  Init=0  Slope=1  Bias=0  DataSize=1  fpDataType=boolean  BlockIOType=Outport  DeviceType=0
  out_OUT_PCAN.Tx_Dig.In_Dig_01_Sts.MessageEnable : KIBES_Signal/KIBES_Signal  MBDS_LibraryBlock=on  DatabaseKey=1499  SignalName=OUT_PCAN.Tx_Dig.In_Dig_01_Sts.MessageEnable  SymbolName=OUT_PCAN_Tx_Dig_In_Dig_01_Sts_MessageEnable_001499  DataType=boolean  Init=0  Slope=1  Bias=0  DataSize=1  fpDataType=boolean  BlockIOType=Outport  DeviceType=0
  out_OUT_PCAN.Tx_Dig.In_Dig_02_Sts.IN_DIG_DIAG : KIBES_Signal/KIBES_Signal  MBDS_LibraryBlock=on  DatabaseKey=1403  SignalName=OUT_PCAN.Tx_Dig.In_Dig_02_Sts.IN_DIG_DIAG  SymbolName=OUT_PCAN_Tx_Dig_In_Dig_02_Sts_IN_DIG_DIAG_001403  DataType=uint16  Init=0  Slope=1  Bias=0  DataSize=1  fpDataType=uint16  BlockIOType=Outport  DeviceType=0
  out_OUT_PCAN.Tx_Dig.In_Dig_02_Sts.IN_DIG_Val : KIBES_Signal/KIBES_Signal  MBDS_LibraryBlock=on  DatabaseKey=1404  SignalName=OUT_PCAN.Tx_Dig.In_Dig_02_Sts.IN_DIG_Val  SymbolName=OUT_PCAN_Tx_Dig_In_Dig_02_Sts_IN_DIG_Val_001404  DataType=boolean  Init=0  Slope=1  Bias=0  DataSize=1  fpDataType=boolean  BlockIOType=Outport  DeviceType=0
  out_OUT_PCAN.Tx_Dig.In_Dig_02_Sts.MessageEnable : KIBES_Signal/KIBES_Signal  MBDS_LibraryBlock=on  DatabaseKey=1500  SignalName=OUT_PCAN.Tx_Dig.In_Dig_02_Sts.MessageEnable  SymbolName=OUT_PCAN_Tx_Dig_In_Dig_02_Sts_MessageEnable_001500  DataType=boolean  Init=0  Slope=1  Bias=0  DataSize=1  fpDataType=boolean  BlockIOType=Outport  DeviceType=0
  out_OUT_PCAN.Tx_Dig.In_Dig_03_Sts.IN_DIG_DIAG : KIBES_Signal/KIBES_Signal  MBDS_LibraryBlock=on  DatabaseKey=1405  SignalName=OUT_PCAN.Tx_Dig.In_Dig_03_Sts.IN_DIG_DIAG  SymbolName=OUT_PCAN_Tx_Dig_In_Dig_03_Sts_IN_DIG_DIAG_001405  DataType=uint16  Init=0  Slope=1  Bias=0  DataSize=1  fpDataType=uint16  BlockIOType=Outport  DeviceType=0
  out_OUT_PCAN.Tx_Dig.In_Dig_03_Sts.IN_DIG_Val : KIBES_Signal/KIBES_Signal  MBDS_LibraryBlock=on  DatabaseKey=1406  SignalName=OUT_PCAN.Tx_Dig.In_Dig_03_Sts.IN_DIG_Val  SymbolName=OUT_PCAN_Tx_Dig_In_Dig_03_Sts_IN_DIG_Val_001406  DataType=boolean  Init=0  Slope=1  Bias=0  DataSize=1  fpDataType=boolean  BlockIOType=Outport  DeviceType=0
  out_OUT_PCAN.Tx_Dig.In_Dig_03_Sts.MessageEnable : KIBES_Signal/KIBES_Signal  MBDS_LibraryBlock=on  DatabaseKey=1501  SignalName=OUT_PCAN.Tx_Dig.In_Dig_03_Sts.MessageEnable  SymbolName=OUT_PCAN_Tx_Dig_In_Dig_03_Sts_MessageEnable_001501  DataType=boolean  Init=0  Slope=1  Bias=0  DataSize=1  fpDataType=boolean  BlockIOType=Outport  DeviceType=0
  out_OUT_PCAN.Tx_Dig.In_Dig_04_Sts.IN_DIG_DIAG : KIBES_Signal/KIBES_Signal  MBDS_LibraryBlock=on  DatabaseKey=1407  SignalName=OUT_PCAN.Tx_Dig.In_Dig_04_Sts.IN_DIG_DIAG  SymbolName=OUT_PCAN_Tx_Dig_In_Dig_04_Sts_IN_DIG_DIAG_001407  DataType=uint16  Init=0  Slope=1  Bias=0  DataSize=1  fpDataType=uint16  BlockIOType=Outport  DeviceType=0
  out_OUT_PCAN.Tx_Dig.In_Dig_04_Sts.IN_DIG_Val : KIBES_Signal/KIBES_Signal  MBDS_LibraryBlock=on  DatabaseKey=1408  SignalName=OUT_PCAN.Tx_Dig.In_Dig_04_Sts.IN_DIG_Val  SymbolName=OUT_PCAN_Tx_Dig_In_Dig_04_Sts_IN_DIG_Val_001408  DataType=boolean  Init=0  Slope=1  Bias=0  DataSize=1  fpDataType=boolean  BlockIOType=Outport  DeviceType=0
  out_OUT_PCAN.Tx_Dig.In_Dig_04_Sts.MessageEnable : KIBES_Signal/KIBES_Signal  MBDS_LibraryBlock=on  DatabaseKey=1502  SignalName=OUT_PCAN.Tx_Dig.In_Dig_04_Sts.MessageEnable  SymbolName=OUT_PCAN_Tx_Dig_In_Dig_04_Sts_MessageEnable_001502  DataType=boolean  Init=0  Slope=1  Bias=0  DataSize=1  fpDataType=boolean  BlockIOType=Outport  DeviceType=0
  out_OUT_PCAN.Tx_Dig.In_Dig_05_Sts.IN_DIG_DIAG : KIBES_Signal/KIBES_Signal  MBDS_LibraryBlock=on  DatabaseKey=1409  SignalName=OUT_PCAN.Tx_Dig.In_Dig_05_Sts.IN_DIG_DIAG  SymbolName=OUT_PCAN_Tx_Dig_In_Dig_05_Sts_IN_DIG_DIAG_001409  DataType=uint16  Init=0  Slope=1  Bias=0  DataSize=1  fpDataType=uint16  BlockIOType=Outport  DeviceType=0
  out_OUT_PCAN.Tx_Dig.In_Dig_05_Sts.IN_DIG_Val : KIBES_Signal/KIBES_Signal  MBDS_LibraryBlock=on  DatabaseKey=1410  SignalName=OUT_PCAN.Tx_Dig.In_Dig_05_Sts.IN_DIG_Val  SymbolName=OUT_PCAN_Tx_Dig_In_Dig_05_Sts_IN_DIG_Val_001410  DataType=boolean  Init=0  Slope=1  Bias=0  DataSize=1  fpDataType=boolean  BlockIOType=Outport  DeviceType=0
  out_OUT_PCAN.Tx_Dig.In_Dig_05_Sts.MessageEnable : KIBES_Signal/KIBES_Signal  MBDS_LibraryBlock=on  DatabaseKey=1793  SignalName=OUT_PCAN.Tx_Dig.In_Dig_05_Sts.MessageEnable  SymbolName=OUT_PCAN_Tx_Dig_In_Dig_05_Sts_MessageEnable_001793  DataType=boolean  Init=0  Slope=1  Bias=0  DataSize=1  fpDataType=boolean  BlockIOType=Outport  DeviceType=0
  out_OUT_PCAN.Tx_Dig.In_Dig_06_Sts.IN_DIG_DIAG : KIBES_Signal/KIBES_Signal  MBDS_LibraryBlock=on  DatabaseKey=1411  SignalName=OUT_PCAN.Tx_Dig.In_Dig_06_Sts.IN_DIG_DIAG  SymbolName=OUT_PCAN_Tx_Dig_In_Dig_06_Sts_IN_DIG_DIAG_001411  DataType=uint16  Init=0  Slope=1  Bias=0  DataSize=1  fpDataType=uint16  BlockIOType=Outport  DeviceType=0
  out_OUT_PCAN.Tx_Dig.In_Dig_06_Sts.IN_DIG_Val : KIBES_Signal/KIBES_Signal  MBDS_LibraryBlock=on  DatabaseKey=1412  SignalName=OUT_PCAN.Tx_Dig.In_Dig_06_Sts.IN_DIG_Val  SymbolName=OUT_PCAN_Tx_Dig_In_Dig_06_Sts_IN_DIG_Val_001412  DataType=boolean  Init=0  Slope=1  Bias=0  DataSize=1  fpDataType=boolean  BlockIOType=Outport  DeviceType=0
  out_OUT_PCAN.Tx_Dig.In_Dig_06_Sts.MessageEnable : KIBES_Signal/KIBES_Signal  MBDS_LibraryBlock=on  DatabaseKey=1503  SignalName=OUT_PCAN.Tx_Dig.In_Dig_06_Sts.MessageEnable  SymbolName=OUT_PCAN_Tx_Dig_In_Dig_06_Sts_MessageEnable_001503  DataType=boolean  Init=0  Slope=1  Bias=0  DataSize=1  fpDataType=boolean  BlockIOType=Outport  DeviceType=0
  out_OUT_PCAN.Tx_Dig.In_Dig_07_Sts.IN_DIG_DIAG : KIBES_Signal/KIBES_Signal  MBDS_LibraryBlock=on  DatabaseKey=1413  SignalName=OUT_PCAN.Tx_Dig.In_Dig_07_Sts.IN_DIG_DIAG  SymbolName=OUT_PCAN_Tx_Dig_In_Dig_07_Sts_IN_DIG_DIAG_001413  DataType=uint16  Init=0  Slope=1  Bias=0  DataSize=1  fpDataType=uint16  BlockIOType=Outport  DeviceType=0
  out_OUT_PCAN.Tx_Dig.In_Dig_07_Sts.IN_DIG_Val : KIBES_Signal/KIBES_Signal  MBDS_LibraryBlock=on  DatabaseKey=1414  SignalName=OUT_PCAN.Tx_Dig.In_Dig_07_Sts.IN_DIG_Val  SymbolName=OUT_PCAN_Tx_Dig_In_Dig_07_Sts_IN_DIG_Val_001414  DataType=boolean  Init=0  Slope=1  Bias=0  DataSize=1  fpDataType=boolean  BlockIOType=Outport  DeviceType=0
  out_OUT_PCAN.Tx_Dig.In_Dig_07_Sts.MessageEnable : KIBES_Signal/KIBES_Signal  MBDS_LibraryBlock=on  DatabaseKey=1794  SignalName=OUT_PCAN.Tx_Dig.In_Dig_07_Sts.MessageEnable  SymbolName=OUT_PCAN_Tx_Dig_In_Dig_07_Sts_MessageEnable_001794  DataType=boolean  Init=0  Slope=1  Bias=0  DataSize=1  fpDataType=boolean  BlockIOType=Outport  DeviceType=0
  out_OUT_PCAN.Tx_Dig.In_Dig_08_Sts.IN_DIG_DIAG : KIBES_Signal/KIBES_Signal  MBDS_LibraryBlock=on  DatabaseKey=1415  SignalName=OUT_PCAN.Tx_Dig.In_Dig_08_Sts.IN_DIG_DIAG  SymbolName=OUT_PCAN_Tx_Dig_In_Dig_08_Sts_IN_DIG_DIAG_001415  DataType=uint16  Init=0  Slope=1  Bias=0  DataSize=1  fpDataType=uint16  BlockIOType=Outport  DeviceType=0
  out_OUT_PCAN.Tx_Dig.In_Dig_08_Sts.IN_DIG_Val : KIBES_Signal/KIBES_Signal  MBDS_LibraryBlock=on  DatabaseKey=1416  SignalName=OUT_PCAN.Tx_Dig.In_Dig_08_Sts.IN_DIG_Val  SymbolName=OUT_PCAN_Tx_Dig_In_Dig_08_Sts_IN_DIG_Val_001416  DataType=boolean  Init=0  Slope=1  Bias=0  DataSize=1  fpDataType=boolean  BlockIOType=Outport  DeviceType=0
  out_OUT_PCAN.Tx_Dig.In_Dig_08_Sts.MessageEnable : KIBES_Signal/KIBES_Signal  MBDS_LibraryBlock=on  DatabaseKey=1795  SignalName=OUT_PCAN.Tx_Dig.In_Dig_08_Sts.MessageEnable  SymbolName=OUT_PCAN_Tx_Dig_In_Dig_08_Sts_MessageEnable_001795  DataType=boolean  Init=0  Slope=1  Bias=0  DataSize=1  fpDataType=boolean  BlockIOType=Outport  DeviceType=0
  out_OUT_PCAN.Tx_Dig.In_Dig_09_Sts.IN_DIG_DIAG : KIBES_Signal/KIBES_Signal  MBDS_LibraryBlock=on  DatabaseKey=1417  SignalName=OUT_PCAN.Tx_Dig.In_Dig_09_Sts.IN_DIG_DIAG  SymbolName=OUT_PCAN_Tx_Dig_In_Dig_09_Sts_IN_DIG_DIAG_001417  DataType=uint16  Init=0  Slope=1  Bias=0  DataSize=1  fpDataType=uint16  BlockIOType=Outport  DeviceType=0
  out_OUT_PCAN.Tx_Dig.In_Dig_09_Sts.IN_DIG_Val : KIBES_Signal/KIBES_Signal  MBDS_LibraryBlock=on  DatabaseKey=1418  SignalName=OUT_PCAN.Tx_Dig.In_Dig_09_Sts.IN_DIG_Val  SymbolName=OUT_PCAN_Tx_Dig_In_Dig_09_Sts_IN_DIG_Val_001418  DataType=boolean  Init=0  Slope=1  Bias=0  DataSize=1  fpDataType=boolean  BlockIOType=Outport  DeviceType=0
  out_OUT_PCAN.Tx_Dig.In_Dig_09_Sts.MessageEnable : KIBES_Signal/KIBES_Signal  MBDS_LibraryBlock=on  DatabaseKey=1796  SignalName=OUT_PCAN.Tx_Dig.In_Dig_09_Sts.MessageEnable  SymbolName=OUT_PCAN_Tx_Dig_In_Dig_09_Sts_MessageEnable_001796  DataType=boolean  Init=0  Slope=1  Bias=0  DataSize=1  fpDataType=boolean  BlockIOType=Outport  DeviceType=0
  out_OUT_PCAN.Tx_Dig.In_Dig_10_Sts.IN_DIG_DIAG : KIBES_Signal/KIBES_Signal  MBDS_LibraryBlock=on  DatabaseKey=1419  SignalName=OUT_PCAN.Tx_Dig.In_Dig_10_Sts.IN_DIG_DIAG  SymbolName=OUT_PCAN_Tx_Dig_In_Dig_10_Sts_IN_DIG_DIAG_001419  DataType=uint16  Init=0  Slope=1  Bias=0  DataSize=1  fpDataType=uint16  BlockIOType=Outport  DeviceType=0
  out_OUT_PCAN.Tx_Dig.In_Dig_10_Sts.IN_DIG_Val : KIBES_Signal/KIBES_Signal  MBDS_LibraryBlock=on  DatabaseKey=1420  SignalName=OUT_PCAN.Tx_Dig.In_Dig_10_Sts.IN_DIG_Val  SymbolName=OUT_PCAN_Tx_Dig_In_Dig_10_Sts_IN_DIG_Val_001420  DataType=boolean  Init=0  Slope=1  Bias=0  DataSize=1  fpDataType=boolean  BlockIOType=Outport  DeviceType=0
  out_OUT_PCAN.Tx_Dig.In_Dig_10_Sts.MessageEnable : KIBES_Signal/KIBES_Signal  MBDS_LibraryBlock=on  DatabaseKey=1797  SignalName=OUT_PCAN.Tx_Dig.In_Dig_10_Sts.MessageEnable  SymbolName=OUT_PCAN_Tx_Dig_In_Dig_10_Sts_MessageEnable_001797  DataType=boolean  Init=0  Slope=1  Bias=0  DataSize=1  fpDataType=boolean  BlockIOType=Outport  DeviceType=0
  out_OUT_PCAN.Tx_Dig.In_Dig_11_Sts.IN_DIG_DIAG : KIBES_Signal/KIBES_Signal  MBDS_LibraryBlock=on  DatabaseKey=1421  SignalName=OUT_PCAN.Tx_Dig.In_Dig_11_Sts.IN_DIG_DIAG  SymbolName=OUT_PCAN_Tx_Dig_In_Dig_11_Sts_IN_DIG_DIAG_001421  DataType=uint16  Init=0  Slope=1  Bias=0  DataSize=1  fpDataType=uint16  BlockIOType=Outport  DeviceType=0
  out_OUT_PCAN.Tx_Dig.In_Dig_11_Sts.IN_DIG_Val : KIBES_Signal/KIBES_Signal  MBDS_LibraryBlock=on  DatabaseKey=1422  SignalName=OUT_PCAN.Tx_Dig.In_Dig_11_Sts.IN_DIG_Val  SymbolName=OUT_PCAN_Tx_Dig_In_Dig_11_Sts_IN_DIG_Val_001422  DataType=boolean  Init=0  Slope=1  Bias=0  DataSize=1  fpDataType=boolean  BlockIOType=Outport  DeviceType=0
  out_OUT_PCAN.Tx_Dig.In_Dig_11_Sts.MessageEnable : KIBES_Signal/KIBES_Signal  MBDS_LibraryBlock=on  DatabaseKey=1504  SignalName=OUT_PCAN.Tx_Dig.In_Dig_11_Sts.MessageEnable  SymbolName=OUT_PCAN_Tx_Dig_In_Dig_11_Sts_MessageEnable_001504  DataType=boolean  Init=0  Slope=1  Bias=0  DataSize=1  fpDataType=boolean  BlockIOType=Outport  DeviceType=0
  out_OUT_PCAN.Tx_Dig.In_Dig_12_Sts.IN_DIG_DIAG : KIBES_Signal/KIBES_Signal  MBDS_LibraryBlock=on  DatabaseKey=1423  SignalName=OUT_PCAN.Tx_Dig.In_Dig_12_Sts.IN_DIG_DIAG  SymbolName=OUT_PCAN_Tx_Dig_In_Dig_12_Sts_IN_DIG_DIAG_001423  DataType=uint16  Init=0  Slope=1  Bias=0  DataSize=1  fpDataType=uint16  BlockIOType=Outport  DeviceType=0
  out_OUT_PCAN.Tx_Dig.In_Dig_12_Sts.IN_DIG_Val : KIBES_Signal/KIBES_Signal  MBDS_LibraryBlock=on  DatabaseKey=1424  SignalName=OUT_PCAN.Tx_Dig.In_Dig_12_Sts.IN_DIG_Val  SymbolName=OUT_PCAN_Tx_Dig_In_Dig_12_Sts_IN_DIG_Val_001424  DataType=boolean  Init=0  Slope=1  Bias=0  DataSize=1  fpDataType=boolean  BlockIOType=Outport  DeviceType=0
  out_OUT_PCAN.Tx_Dig.In_Dig_12_Sts.MessageEnable : KIBES_Signal/KIBES_Signal  MBDS_LibraryBlock=on  DatabaseKey=1798  SignalName=OUT_PCAN.Tx_Dig.In_Dig_12_Sts.MessageEnable  SymbolName=OUT_PCAN_Tx_Dig_In_Dig_12_Sts_MessageEnable_001798  DataType=boolean  Init=0  Slope=1  Bias=0  DataSize=1  fpDataType=boolean  BlockIOType=Outport  DeviceType=0
  out_OUT_PCAN.Tx_Dig.In_Dig_13_Sts.IN_DIG_DIAG : KIBES_Signal/KIBES_Signal  MBDS_LibraryBlock=on  DatabaseKey=1425  SignalName=OUT_PCAN.Tx_Dig.In_Dig_13_Sts.IN_DIG_DIAG  SymbolName=OUT_PCAN_Tx_Dig_In_Dig_13_Sts_IN_DIG_DIAG_001425  DataType=uint16  Init=0  Slope=1  Bias=0  DataSize=1  fpDataType=uint16  BlockIOType=Outport  DeviceType=0
  out_OUT_PCAN.Tx_Dig.In_Dig_13_Sts.IN_DIG_Val : KIBES_Signal/KIBES_Signal  MBDS_LibraryBlock=on  DatabaseKey=1426  SignalName=OUT_PCAN.Tx_Dig.In_Dig_13_Sts.IN_DIG_Val  SymbolName=OUT_PCAN_Tx_Dig_In_Dig_13_Sts_IN_DIG_Val_001426  DataType=boolean  Init=0  Slope=1  Bias=0  DataSize=1  fpDataType=boolean  BlockIOType=Outport  DeviceType=0
  out_OUT_PCAN.Tx_Dig.In_Dig_13_Sts.MessageEnable : KIBES_Signal/KIBES_Signal  MBDS_LibraryBlock=on  DatabaseKey=1505  SignalName=OUT_PCAN.Tx_Dig.In_Dig_13_Sts.MessageEnable  SymbolName=OUT_PCAN_Tx_Dig_In_Dig_13_Sts_MessageEnable_001505  DataType=boolean  Init=0  Slope=1  Bias=0  DataSize=1  fpDataType=boolean  BlockIOType=Outport  DeviceType=0
  out_OUT_PCAN.Tx_Dig.In_Dig_14_Sts.IN_DIG_DIAG : KIBES_Signal/KIBES_Signal  MBDS_LibraryBlock=on  DatabaseKey=1427  SignalName=OUT_PCAN.Tx_Dig.In_Dig_14_Sts.IN_DIG_DIAG  SymbolName=OUT_PCAN_Tx_Dig_In_Dig_14_Sts_IN_DIG_DIAG_001427  DataType=uint16  Init=0  Slope=1  Bias=0  DataSize=1  fpDataType=uint16  BlockIOType=Outport  DeviceType=0
  out_OUT_PCAN.Tx_Dig.In_Dig_14_Sts.IN_DIG_Val : KIBES_Signal/KIBES_Signal  MBDS_LibraryBlock=on  DatabaseKey=1428  SignalName=OUT_PCAN.Tx_Dig.In_Dig_14_Sts.IN_DIG_Val  SymbolName=OUT_PCAN_Tx_Dig_In_Dig_14_Sts_IN_DIG_Val_001428  DataType=boolean  Init=0  Slope=1  Bias=0  DataSize=1  fpDataType=boolean  BlockIOType=Outport  DeviceType=0
  out_OUT_PCAN.Tx_Dig.In_Dig_14_Sts.MessageEnable : KIBES_Signal/KIBES_Signal  MBDS_LibraryBlock=on  DatabaseKey=1506  SignalName=OUT_PCAN.Tx_Dig.In_Dig_14_Sts.MessageEnable  SymbolName=OUT_PCAN_Tx_Dig_In_Dig_14_Sts_MessageEnable_001506  DataType=boolean  Init=0  Slope=1  Bias=0  DataSize=1  fpDataType=boolean  BlockIOType=Outport  DeviceType=0
  out_OUT_PCAN.Tx_Dig.In_Dig_15_Sts.IN_DIG_DIAG : KIBES_Signal/KIBES_Signal  MBDS_LibraryBlock=on  DatabaseKey=1429  SignalName=OUT_PCAN.Tx_Dig.In_Dig_15_Sts.IN_DIG_DIAG  SymbolName=OUT_PCAN_Tx_Dig_In_Dig_15_Sts_IN_DIG_DIAG_001429  DataType=uint16  Init=0  Slope=1  Bias=0  DataSize=1  fpDataType=uint16  BlockIOType=Outport  DeviceType=0
  out_OUT_PCAN.Tx_Dig.In_Dig_15_Sts.IN_DIG_Val : KIBES_Signal/KIBES_Signal  MBDS_LibraryBlock=on  DatabaseKey=1430  SignalName=OUT_PCAN.Tx_Dig.In_Dig_15_Sts.IN_DIG_Val  SymbolName=OUT_PCAN_Tx_Dig_In_Dig_15_Sts_IN_DIG_Val_001430  DataType=boolean  Init=0  Slope=1  Bias=0  DataSize=1  fpDataType=boolean  BlockIOType=Outport  DeviceType=0
  out_OUT_PCAN.Tx_Dig.In_Dig_15_Sts.MessageEnable : KIBES_Signal/KIBES_Signal  MBDS_LibraryBlock=on  DatabaseKey=1507  SignalName=OUT_PCAN.Tx_Dig.In_Dig_15_Sts.MessageEnable  SymbolName=OUT_PCAN_Tx_Dig_In_Dig_15_Sts_MessageEnable_001507  DataType=boolean  Init=0  Slope=1  Bias=0  DataSize=1  fpDataType=boolean  BlockIOType=Outport  DeviceType=0
  out_OUT_PCAN.Tx_Dig.In_Dig_16_Sts.IN_DIG_DIAG : KIBES_Signal/KIBES_Signal  MBDS_LibraryBlock=on  DatabaseKey=1431  SignalName=OUT_PCAN.Tx_Dig.In_Dig_16_Sts.IN_DIG_DIAG  SymbolName=OUT_PCAN_Tx_Dig_In_Dig_16_Sts_IN_DIG_DIAG_001431  DataType=uint16  Init=0  Slope=1  Bias=0  DataSize=1  fpDataType=uint16  BlockIOType=Outport  DeviceType=0
  out_OUT_PCAN.Tx_Dig.In_Dig_16_Sts.IN_DIG_Val : KIBES_Signal/KIBES_Signal  MBDS_LibraryBlock=on  DatabaseKey=1432  SignalName=OUT_PCAN.Tx_Dig.In_Dig_16_Sts.IN_DIG_Val  SymbolName=OUT_PCAN_Tx_Dig_In_Dig_16_Sts_IN_DIG_Val_001432  DataType=boolean  Init=0  Slope=1  Bias=0  DataSize=1  fpDataType=boolean  BlockIOType=Outport  DeviceType=0
  out_OUT_PCAN.Tx_Dig.In_Dig_16_Sts.MessageEnable : KIBES_Signal/KIBES_Signal  MBDS_LibraryBlock=on  DatabaseKey=1508  SignalName=OUT_PCAN.Tx_Dig.In_Dig_16_Sts.MessageEnable  SymbolName=OUT_PCAN_Tx_Dig_In_Dig_16_Sts_MessageEnable_001508  DataType=boolean  Init=0  Slope=1  Bias=0  DataSize=1  fpDataType=boolean  BlockIOType=Outport  DeviceType=0
  out_OUT_PCAN.Tx_Dig.In_Dig_17_Sts.IN_DIG_DIAG : KIBES_Signal/KIBES_Signal  MBDS_LibraryBlock=on  DatabaseKey=1433  SignalName=OUT_PCAN.Tx_Dig.In_Dig_17_Sts.IN_DIG_DIAG  SymbolName=OUT_PCAN_Tx_Dig_In_Dig_17_Sts_IN_DIG_DIAG_001433  DataType=uint16  Init=0  Slope=1  Bias=0  DataSize=1  fpDataType=uint16  BlockIOType=Outport  DeviceType=0
  out_OUT_PCAN.Tx_Dig.In_Dig_17_Sts.IN_DIG_Val : KIBES_Signal/KIBES_Signal  MBDS_LibraryBlock=on  DatabaseKey=1434  SignalName=OUT_PCAN.Tx_Dig.In_Dig_17_Sts.IN_DIG_Val  SymbolName=OUT_PCAN_Tx_Dig_In_Dig_17_Sts_IN_DIG_Val_001434  DataType=boolean  Init=0  Slope=1  Bias=0  DataSize=1  fpDataType=boolean  BlockIOType=Outport  DeviceType=0
  out_OUT_PCAN.Tx_Dig.In_Dig_17_Sts.MessageEnable : KIBES_Signal/KIBES_Signal  MBDS_LibraryBlock=on  DatabaseKey=1509  SignalName=OUT_PCAN.Tx_Dig.In_Dig_17_Sts.MessageEnable  SymbolName=OUT_PCAN_Tx_Dig_In_Dig_17_Sts_MessageEnable_001509  DataType=boolean  Init=0  Slope=1  Bias=0  DataSize=1  fpDataType=boolean  BlockIOType=Outport  DeviceType=0
  out_OUT_PCAN.Tx_Dig.In_Dig_18_Sts.IN_DIG_DIAG : KIBES_Signal/KIBES_Signal  MBDS_LibraryBlock=on  DatabaseKey=1435  SignalName=OUT_PCAN.Tx_Dig.In_Dig_18_Sts.IN_DIG_DIAG  SymbolName=OUT_PCAN_Tx_Dig_In_Dig_18_Sts_IN_DIG_DIAG_001435  DataType=uint16  Init=0  Slope=1  Bias=0  DataSize=1  fpDataType=uint16  BlockIOType=Outport  DeviceType=0
  out_OUT_PCAN.Tx_Dig.In_Dig_18_Sts.IN_DIG_Val : KIBES_Signal/KIBES_Signal  MBDS_LibraryBlock=on  DatabaseKey=1436  SignalName=OUT_PCAN.Tx_Dig.In_Dig_18_Sts.IN_DIG_Val  SymbolName=OUT_PCAN_Tx_Dig_In_Dig_18_Sts_IN_DIG_Val_001436  DataType=boolean  Init=0  Slope=1  Bias=0  DataSize=1  fpDataType=boolean  BlockIOType=Outport  DeviceType=0
  out_OUT_PCAN.Tx_Dig.In_Dig_18_Sts.MessageEnable : KIBES_Signal/KIBES_Signal  MBDS_LibraryBlock=on  DatabaseKey=1510  SignalName=OUT_PCAN.Tx_Dig.In_Dig_18_Sts.MessageEnable  SymbolName=OUT_PCAN_Tx_Dig_In_Dig_18_Sts_MessageEnable_001510  DataType=boolean  Init=0  Slope=1  Bias=0  DataSize=1  fpDataType=boolean  BlockIOType=Outport  DeviceType=0
  out_OUT_PCAN.Tx_Dig.In_Dig_19_Sts.IN_DIG_DIAG : KIBES_Signal/KIBES_Signal  MBDS_LibraryBlock=on  DatabaseKey=1437  SignalName=OUT_PCAN.Tx_Dig.In_Dig_19_Sts.IN_DIG_DIAG  SymbolName=OUT_PCAN_Tx_Dig_In_Dig_19_Sts_IN_DIG_DIAG_001437  DataType=uint16  Init=0  Slope=1  Bias=0  DataSize=1  fpDataType=uint16  BlockIOType=Outport  DeviceType=0
  out_OUT_PCAN.Tx_Dig.In_Dig_19_Sts.IN_DIG_Val : KIBES_Signal/KIBES_Signal  MBDS_LibraryBlock=on  DatabaseKey=1438  SignalName=OUT_PCAN.Tx_Dig.In_Dig_19_Sts.IN_DIG_Val  SymbolName=OUT_PCAN_Tx_Dig_In_Dig_19_Sts_IN_DIG_Val_001438  DataType=boolean  Init=0  Slope=1  Bias=0  DataSize=1  fpDataType=boolean  BlockIOType=Outport  DeviceType=0
  out_OUT_PCAN.Tx_Dig.In_Dig_19_Sts.MessageEnable : KIBES_Signal/KIBES_Signal  MBDS_LibraryBlock=on  DatabaseKey=1511  SignalName=OUT_PCAN.Tx_Dig.In_Dig_19_Sts.MessageEnable  SymbolName=OUT_PCAN_Tx_Dig_In_Dig_19_Sts_MessageEnable_001511  DataType=boolean  Init=0  Slope=1  Bias=0  DataSize=1  fpDataType=boolean  BlockIOType=Outport  DeviceType=0
  out_OUT_PCAN.Tx_Dig.In_Dig_20_Sts.IN_DIG_DIAG : KIBES_Signal/KIBES_Signal  MBDS_LibraryBlock=on  DatabaseKey=1439  SignalName=OUT_PCAN.Tx_Dig.In_Dig_20_Sts.IN_DIG_DIAG  SymbolName=OUT_PCAN_Tx_Dig_In_Dig_20_Sts_IN_DIG_DIAG_001439  DataType=uint16  Init=0  Slope=1  Bias=0  DataSize=1  fpDataType=uint16  BlockIOType=Outport  DeviceType=0
  out_OUT_PCAN.Tx_Dig.In_Dig_20_Sts.IN_DIG_Val : KIBES_Signal/KIBES_Signal  MBDS_LibraryBlock=on  DatabaseKey=1440  SignalName=OUT_PCAN.Tx_Dig.In_Dig_20_Sts.IN_DIG_Val  SymbolName=OUT_PCAN_Tx_Dig_In_Dig_20_Sts_IN_DIG_Val_001440  DataType=boolean  Init=0  Slope=1  Bias=0  DataSize=1  fpDataType=boolean  BlockIOType=Outport  DeviceType=0
  out_OUT_PCAN.Tx_Dig.In_Dig_20_Sts.MessageEnable : KIBES_Signal/KIBES_Signal  MBDS_LibraryBlock=on  DatabaseKey=1512  SignalName=OUT_PCAN.Tx_Dig.In_Dig_20_Sts.MessageEnable  SymbolName=OUT_PCAN_Tx_Dig_In_Dig_20_Sts_MessageEnable_001512  DataType=boolean  Init=0  Slope=1  Bias=0  DataSize=1  fpDataType=boolean  BlockIOType=Outport  DeviceType=0
  out_OUT_PCAN.Tx_Dig.In_Dig_21_Sts.IN_DIG_DIAG : KIBES_Signal/KIBES_Signal  MBDS_LibraryBlock=on  DatabaseKey=1441  SignalName=OUT_PCAN.Tx_Dig.In_Dig_21_Sts.IN_DIG_DIAG  SymbolName=OUT_PCAN_Tx_Dig_In_Dig_21_Sts_IN_DIG_DIAG_001441  DataType=uint16  Init=0  Slope=1  Bias=0  DataSize=1  fpDataType=uint16  BlockIOType=Outport  DeviceType=0
  out_OUT_PCAN.Tx_Dig.In_Dig_21_Sts.IN_DIG_Val : KIBES_Signal/KIBES_Signal  MBDS_LibraryBlock=on  DatabaseKey=1442  SignalName=OUT_PCAN.Tx_Dig.In_Dig_21_Sts.IN_DIG_Val  SymbolName=OUT_PCAN_Tx_Dig_In_Dig_21_Sts_IN_DIG_Val_001442  DataType=boolean  Init=0  Slope=1  Bias=0  DataSize=1  fpDataType=boolean  BlockIOType=Outport  DeviceType=0
  out_OUT_PCAN.Tx_Dig.In_Dig_21_Sts.MessageEnable : KIBES_Signal/KIBES_Signal  MBDS_LibraryBlock=on  DatabaseKey=1513  SignalName=OUT_PCAN.Tx_Dig.In_Dig_21_Sts.MessageEnable  SymbolName=OUT_PCAN_Tx_Dig_In_Dig_21_Sts_MessageEnable_001513  DataType=boolean  Init=0  Slope=1  Bias=0  DataSize=1  fpDataType=boolean  BlockIOType=Outport  DeviceType=0
  out_OUT_PCAN.Tx_Dig.In_Dig_22_Sts.IN_DIG_DIAG : KIBES_Signal/KIBES_Signal  MBDS_LibraryBlock=on  DatabaseKey=1443  SignalName=OUT_PCAN.Tx_Dig.In_Dig_22_Sts.IN_DIG_DIAG  SymbolName=OUT_PCAN_Tx_Dig_In_Dig_22_Sts_IN_DIG_DIAG_001443  DataType=uint16  Init=0  Slope=1  Bias=0  DataSize=1  fpDataType=uint16  BlockIOType=Outport  DeviceType=0
  out_OUT_PCAN.Tx_Dig.In_Dig_22_Sts.IN_DIG_Val : KIBES_Signal/KIBES_Signal  MBDS_LibraryBlock=on  DatabaseKey=1444  SignalName=OUT_PCAN.Tx_Dig.In_Dig_22_Sts.IN_DIG_Val  SymbolName=OUT_PCAN_Tx_Dig_In_Dig_22_Sts_IN_DIG_Val_001444  DataType=boolean  Init=0  Slope=1  Bias=0  DataSize=1  fpDataType=boolean  BlockIOType=Outport  DeviceType=0
  out_OUT_PCAN.Tx_Dig.In_Dig_22_Sts.MessageEnable : KIBES_Signal/KIBES_Signal  MBDS_LibraryBlock=on  DatabaseKey=1799  SignalName=OUT_PCAN.Tx_Dig.In_Dig_22_Sts.MessageEnable  SymbolName=OUT_PCAN_Tx_Dig_In_Dig_22_Sts_MessageEnable_001799  DataType=boolean  Init=0  Slope=1  Bias=0  DataSize=1  fpDataType=boolean  BlockIOType=Outport  DeviceType=0
  out_OUT_PCAN.Tx_Dig.In_Dig_23_Sts.IN_DIG_DIAG : KIBES_Signal/KIBES_Signal  MBDS_LibraryBlock=on  DatabaseKey=1445  SignalName=OUT_PCAN.Tx_Dig.In_Dig_23_Sts.IN_DIG_DIAG  SymbolName=OUT_PCAN_Tx_Dig_In_Dig_23_Sts_IN_DIG_DIAG_001445  DataType=uint16  Init=0  Slope=1  Bias=0  DataSize=1  fpDataType=uint16  BlockIOType=Outport  DeviceType=0
  out_OUT_PCAN.Tx_Dig.In_Dig_23_Sts.IN_DIG_Val : KIBES_Signal/KIBES_Signal  MBDS_LibraryBlock=on  DatabaseKey=1446  SignalName=OUT_PCAN.Tx_Dig.In_Dig_23_Sts.IN_DIG_Val  SymbolName=OUT_PCAN_Tx_Dig_In_Dig_23_Sts_IN_DIG_Val_001446  DataType=boolean  Init=0  Slope=1  Bias=0  DataSize=1  fpDataType=boolean  BlockIOType=Outport  DeviceType=0
  out_OUT_PCAN.Tx_Dig.In_Dig_23_Sts.MessageEnable : KIBES_Signal/KIBES_Signal  MBDS_LibraryBlock=on  DatabaseKey=1800  SignalName=OUT_PCAN.Tx_Dig.In_Dig_23_Sts.MessageEnable  SymbolName=OUT_PCAN_Tx_Dig_In_Dig_23_Sts_MessageEnable_001800  DataType=boolean  Init=0  Slope=1  Bias=0  DataSize=1  fpDataType=boolean  BlockIOType=Outport  DeviceType=0
  out_OUT_PCAN.Tx_Dig.In_Dig_24_Sts.IN_DIG_DIAG : KIBES_Signal/KIBES_Signal  MBDS_LibraryBlock=on  DatabaseKey=1447  SignalName=OUT_PCAN.Tx_Dig.In_Dig_24_Sts.IN_DIG_DIAG  SymbolName=OUT_PCAN_Tx_Dig_In_Dig_24_Sts_IN_DIG_DIAG_001447  DataType=uint16  Init=0  Slope=1  Bias=0  DataSize=1  fpDataType=uint16  BlockIOType=Outport  DeviceType=0
  out_OUT_PCAN.Tx_Dig.In_Dig_24_Sts.IN_DIG_Val : KIBES_Signal/KIBES_Signal  MBDS_LibraryBlock=on  DatabaseKey=1448  SignalName=OUT_PCAN.Tx_Dig.In_Dig_24_Sts.IN_DIG_Val  SymbolName=OUT_PCAN_Tx_Dig_In_Dig_24_Sts_IN_DIG_Val_001448  DataType=boolean  Init=0  Slope=1  Bias=0  DataSize=1  fpDataType=boolean  BlockIOType=Outport  DeviceType=0
  out_OUT_PCAN.Tx_Dig.In_Dig_24_Sts.MessageEnable : KIBES_Signal/KIBES_Signal  MBDS_LibraryBlock=on  DatabaseKey=1515  SignalName=OUT_PCAN.Tx_Dig.In_Dig_24_Sts.MessageEnable  SymbolName=OUT_PCAN_Tx_Dig_In_Dig_24_Sts_MessageEnable_001515  DataType=boolean  Init=0  Slope=1  Bias=0  DataSize=1  fpDataType=boolean  BlockIOType=Outport  DeviceType=0
  out_OUT_PCAN.Tx_Dig.In_Dig_25_Sts.IN_DIG_DIAG : KIBES_Signal/KIBES_Signal  MBDS_LibraryBlock=on  DatabaseKey=1449  SignalName=OUT_PCAN.Tx_Dig.In_Dig_25_Sts.IN_DIG_DIAG  SymbolName=OUT_PCAN_Tx_Dig_In_Dig_25_Sts_IN_DIG_DIAG_001449  DataType=uint16  Init=0  Slope=1  Bias=0  DataSize=1  fpDataType=uint16  BlockIOType=Outport  DeviceType=0
  out_OUT_PCAN.Tx_Dig.In_Dig_25_Sts.IN_DIG_Val : KIBES_Signal/KIBES_Signal  MBDS_LibraryBlock=on  DatabaseKey=1450  SignalName=OUT_PCAN.Tx_Dig.In_Dig_25_Sts.IN_DIG_Val  SymbolName=OUT_PCAN_Tx_Dig_In_Dig_25_Sts_IN_DIG_Val_001450  DataType=boolean  Init=0  Slope=1  Bias=0  DataSize=1  fpDataType=boolean  BlockIOType=Outport  DeviceType=0
  out_OUT_PCAN.Tx_Dig.In_Dig_25_Sts.MessageEnable : KIBES_Signal/KIBES_Signal  MBDS_LibraryBlock=on  DatabaseKey=1514  SignalName=OUT_PCAN.Tx_Dig.In_Dig_25_Sts.MessageEnable  SymbolName=OUT_PCAN_Tx_Dig_In_Dig_25_Sts_MessageEnable_001514  DataType=boolean  Init=0  Slope=1  Bias=0  DataSize=1  fpDataType=boolean  BlockIOType=Outport  DeviceType=0
  out_OUT_PCAN.Tx_Dig.In_Dig_26_Sts.IN_DIG_DIAG : KIBES_Signal/KIBES_Signal  MBDS_LibraryBlock=on  DatabaseKey=1451  SignalName=OUT_PCAN.Tx_Dig.In_Dig_26_Sts.IN_DIG_DIAG  SymbolName=OUT_PCAN_Tx_Dig_In_Dig_26_Sts_IN_DIG_DIAG_001451  DataType=uint16  Init=0  Slope=1  Bias=0  DataSize=1  fpDataType=uint16  BlockIOType=Outport  DeviceType=0
  out_OUT_PCAN.Tx_Dig.In_Dig_26_Sts.IN_DIG_Val : KIBES_Signal/KIBES_Signal  MBDS_LibraryBlock=on  DatabaseKey=1452  SignalName=OUT_PCAN.Tx_Dig.In_Dig_26_Sts.IN_DIG_Val  SymbolName=OUT_PCAN_Tx_Dig_In_Dig_26_Sts_IN_DIG_Val_001452  DataType=boolean  Init=0  Slope=1  Bias=0  DataSize=1  fpDataType=boolean  BlockIOType=Outport  DeviceType=0
  out_OUT_PCAN.Tx_Dig.In_Dig_26_Sts.MessageEnable : KIBES_Signal/KIBES_Signal  MBDS_LibraryBlock=on  DatabaseKey=1516  SignalName=OUT_PCAN.Tx_Dig.In_Dig_26_Sts.MessageEnable  SymbolName=OUT_PCAN_Tx_Dig_In_Dig_26_Sts_MessageEnable_001516  DataType=boolean  Init=0  Slope=1  Bias=0  DataSize=1  fpDataType=boolean  BlockIOType=Outport  DeviceType=0
  out_OUT_PCAN.Tx_Dig.In_Dig_27_Sts.IN_DIG_DIAG : KIBES_Signal/KIBES_Signal  MBDS_LibraryBlock=on  DatabaseKey=1453  SignalName=OUT_PCAN.Tx_Dig.In_Dig_27_Sts.IN_DIG_DIAG  SymbolName=OUT_PCAN_Tx_Dig_In_Dig_27_Sts_IN_DIG_DIAG_001453  DataType=uint16  Init=0  Slope=1  Bias=0  DataSize=1  fpDataType=uint16  BlockIOType=Outport  DeviceType=0
  out_OUT_PCAN.Tx_Dig.In_Dig_27_Sts.IN_DIG_Val : KIBES_Signal/KIBES_Signal  MBDS_LibraryBlock=on  DatabaseKey=1454  SignalName=OUT_PCAN.Tx_Dig.In_Dig_27_Sts.IN_DIG_Val  SymbolName=OUT_PCAN_Tx_Dig_In_Dig_27_Sts_IN_DIG_Val_001454  DataType=boolean  Init=0  Slope=1  Bias=0  DataSize=1  fpDataType=boolean  BlockIOType=Outport  DeviceType=0
  out_OUT_PCAN.Tx_Dig.In_Dig_27_Sts.MessageEnable : KIBES_Signal/KIBES_Signal  MBDS_LibraryBlock=on  DatabaseKey=1517  SignalName=OUT_PCAN.Tx_Dig.In_Dig_27_Sts.MessageEnable  SymbolName=OUT_PCAN_Tx_Dig_In_Dig_27_Sts_MessageEnable_001517  DataType=boolean  Init=0  Slope=1  Bias=0  DataSize=1  fpDataType=boolean  BlockIOType=Outport  DeviceType=0
  out_OUT_PCAN.Tx_Dig.In_Dig_28_Sts.IN_DIG_DIAG : KIBES_Signal/KIBES_Signal  MBDS_LibraryBlock=on  DatabaseKey=1455  SignalName=OUT_PCAN.Tx_Dig.In_Dig_28_Sts.IN_DIG_DIAG  SymbolName=OUT_PCAN_Tx_Dig_In_Dig_28_Sts_IN_DIG_DIAG_001455  DataType=uint16  Init=0  Slope=1  Bias=0  DataSize=1  fpDataType=uint16  BlockIOType=Outport  DeviceType=0
  out_OUT_PCAN.Tx_Dig.In_Dig_28_Sts.IN_DIG_Val : KIBES_Signal/KIBES_Signal  MBDS_LibraryBlock=on  DatabaseKey=1456  SignalName=OUT_PCAN.Tx_Dig.In_Dig_28_Sts.IN_DIG_Val  SymbolName=OUT_PCAN_Tx_Dig_In_Dig_28_Sts_IN_DIG_Val_001456  DataType=boolean  Init=0  Slope=1  Bias=0  DataSize=1  fpDataType=boolean  BlockIOType=Outport  DeviceType=0
  out_OUT_PCAN.Tx_Dig.In_Dig_28_Sts.MessageEnable : KIBES_Signal/KIBES_Signal  MBDS_LibraryBlock=on  DatabaseKey=1518  SignalName=OUT_PCAN.Tx_Dig.In_Dig_28_Sts.MessageEnable  SymbolName=OUT_PCAN_Tx_Dig_In_Dig_28_Sts_MessageEnable_001518  DataType=boolean  Init=0  Slope=1  Bias=0  DataSize=1  fpDataType=boolean  BlockIOType=Outport  DeviceType=0
  out_OUT_PCAN.Tx_Dig.In_Dig_29_Sts.IN_DIG_DIAG : KIBES_Signal/KIBES_Signal  MBDS_LibraryBlock=on  DatabaseKey=1457  SignalName=OUT_PCAN.Tx_Dig.In_Dig_29_Sts.IN_DIG_DIAG  SymbolName=OUT_PCAN_Tx_Dig_In_Dig_29_Sts_IN_DIG_DIAG_001457  DataType=uint16  Init=0  Slope=1  Bias=0  DataSize=1  fpDataType=uint16  BlockIOType=Outport  DeviceType=0
  out_OUT_PCAN.Tx_Dig.In_Dig_29_Sts.IN_DIG_Val : KIBES_Signal/KIBES_Signal  MBDS_LibraryBlock=on  DatabaseKey=1458  SignalName=OUT_PCAN.Tx_Dig.In_Dig_29_Sts.IN_DIG_Val  SymbolName=OUT_PCAN_Tx_Dig_In_Dig_29_Sts_IN_DIG_Val_001458  DataType=boolean  Init=0  Slope=1  Bias=0  DataSize=1  fpDataType=boolean  BlockIOType=Outport  DeviceType=0
  out_OUT_PCAN.Tx_Dig.In_Dig_29_Sts.MessageEnable : KIBES_Signal/KIBES_Signal  MBDS_LibraryBlock=on  DatabaseKey=1519  SignalName=OUT_PCAN.Tx_Dig.In_Dig_29_Sts.MessageEnable  SymbolName=OUT_PCAN_Tx_Dig_In_Dig_29_Sts_MessageEnable_001519  DataType=boolean  Init=0  Slope=1  Bias=0  DataSize=1  fpDataType=boolean  BlockIOType=Outport  DeviceType=0
  out_OUT_PCAN.Tx_Dig.In_Dig_30_Sts.IN_DIG_DIAG : KIBES_Signal/KIBES_Signal  MBDS_LibraryBlock=on  DatabaseKey=1459  SignalName=OUT_PCAN.Tx_Dig.In_Dig_30_Sts.IN_DIG_DIAG  SymbolName=OUT_PCAN_Tx_Dig_In_Dig_30_Sts_IN_DIG_DIAG_001459  DataType=uint16  Init=0  Slope=1  Bias=0  DataSize=1  fpDataType=uint16  BlockIOType=Outport  DeviceType=0
  out_OUT_PCAN.Tx_Dig.In_Dig_30_Sts.IN_DIG_Val : KIBES_Signal/KIBES_Signal  MBDS_LibraryBlock=on  DatabaseKey=1460  SignalName=OUT_PCAN.Tx_Dig.In_Dig_30_Sts.IN_DIG_Val  SymbolName=OUT_PCAN_Tx_Dig_In_Dig_30_Sts_IN_DIG_Val_001460  DataType=boolean  Init=0  Slope=1  Bias=0  DataSize=1  fpDataType=boolean  BlockIOType=Outport  DeviceType=0
  out_OUT_PCAN.Tx_Dig.In_Dig_30_Sts.MessageEnable : KIBES_Signal/KIBES_Signal  MBDS_LibraryBlock=on  DatabaseKey=1520  SignalName=OUT_PCAN.Tx_Dig.In_Dig_30_Sts.MessageEnable  SymbolName=OUT_PCAN_Tx_Dig_In_Dig_30_Sts_MessageEnable_001520  DataType=boolean  Init=0  Slope=1  Bias=0  DataSize=1  fpDataType=boolean  BlockIOType=Outport  DeviceType=0
  out_OUT_PCAN.Tx_Dig.In_Dig_31_Sts.IN_DIG_DIAG : KIBES_Signal/KIBES_Signal  MBDS_LibraryBlock=on  DatabaseKey=1461  SignalName=OUT_PCAN.Tx_Dig.In_Dig_31_Sts.IN_DIG_DIAG  SymbolName=OUT_PCAN_Tx_Dig_In_Dig_31_Sts_IN_DIG_DIAG_001461  DataType=uint16  Init=0  Slope=1  Bias=0  DataSize=1  fpDataType=uint16  BlockIOType=Outport  DeviceType=0
  out_OUT_PCAN.Tx_Dig.In_Dig_31_Sts.IN_DIG_Val : KIBES_Signal/KIBES_Signal  MBDS_LibraryBlock=on  DatabaseKey=1462  SignalName=OUT_PCAN.Tx_Dig.In_Dig_31_Sts.IN_DIG_Val  SymbolName=OUT_PCAN_Tx_Dig_In_Dig_31_Sts_IN_DIG_Val_001462  DataType=boolean  Init=0  Slope=1  Bias=0  DataSize=1  fpDataType=boolean  BlockIOType=Outport  DeviceType=0
  out_OUT_PCAN.Tx_Dig.In_Dig_31_Sts.MessageEnable : KIBES_Signal/KIBES_Signal  MBDS_LibraryBlock=on  DatabaseKey=1521  SignalName=OUT_PCAN.Tx_Dig.In_Dig_31_Sts.MessageEnable  SymbolName=OUT_PCAN_Tx_Dig_In_Dig_31_Sts_MessageEnable_001521  DataType=boolean  Init=0  Slope=1  Bias=0  DataSize=1  fpDataType=boolean  BlockIOType=Outport  DeviceType=0
  out_OUT_PCAN.Tx_Dig.In_Dig_32_Sts.IN_DIG_DIAG : KIBES_Signal/KIBES_Signal  MBDS_LibraryBlock=on  DatabaseKey=1463  SignalName=OUT_PCAN.Tx_Dig.In_Dig_32_Sts.IN_DIG_DIAG  SymbolName=OUT_PCAN_Tx_Dig_In_Dig_32_Sts_IN_DIG_DIAG_001463  DataType=uint16  Init=0  Slope=1  Bias=0  DataSize=1  fpDataType=uint16  BlockIOType=Outport  DeviceType=0
  out_OUT_PCAN.Tx_Dig.In_Dig_32_Sts.IN_DIG_Val : KIBES_Signal/KIBES_Signal  MBDS_LibraryBlock=on  DatabaseKey=1464  SignalName=OUT_PCAN.Tx_Dig.In_Dig_32_Sts.IN_DIG_Val  SymbolName=OUT_PCAN_Tx_Dig_In_Dig_32_Sts_IN_DIG_Val_001464  DataType=boolean  Init=0  Slope=1  Bias=0  DataSize=1  fpDataType=boolean  BlockIOType=Outport  DeviceType=0
  out_OUT_PCAN.Tx_Dig.In_Dig_32_Sts.MessageEnable : KIBES_Signal/KIBES_Signal  MBDS_LibraryBlock=on  DatabaseKey=1522  SignalName=OUT_PCAN.Tx_Dig.In_Dig_32_Sts.MessageEnable  SymbolName=OUT_PCAN_Tx_Dig_In_Dig_32_Sts_MessageEnable_001522  DataType=boolean  Init=0  Slope=1  Bias=0  DataSize=1  fpDataType=boolean  BlockIOType=Outport  DeviceType=0
  out_OUT_PCAN.Tx_Dig.In_Dig_33_Sts.IN_DIG_DIAG : KIBES_Signal/KIBES_Signal  MBDS_LibraryBlock=on  DatabaseKey=1465  SignalName=OUT_PCAN.Tx_Dig.In_Dig_33_Sts.IN_DIG_DIAG  SymbolName=OUT_PCAN_Tx_Dig_In_Dig_33_Sts_IN_DIG_DIAG_001465  DataType=uint16  Init=0  Slope=1  Bias=0  DataSize=1  fpDataType=uint16  BlockIOType=Outport  DeviceType=0
  out_OUT_PCAN.Tx_Dig.In_Dig_33_Sts.IN_DIG_Val : KIBES_Signal/KIBES_Signal  MBDS_LibraryBlock=on  DatabaseKey=1466  SignalName=OUT_PCAN.Tx_Dig.In_Dig_33_Sts.IN_DIG_Val  SymbolName=OUT_PCAN_Tx_Dig_In_Dig_33_Sts_IN_DIG_Val_001466  DataType=boolean  Init=0  Slope=1  Bias=0  DataSize=1  fpDataType=boolean  BlockIOType=Outport  DeviceType=0
  out_OUT_PCAN.Tx_Dig.In_Dig_33_Sts.MessageEnable : KIBES_Signal/KIBES_Signal  MBDS_LibraryBlock=on  DatabaseKey=1523  SignalName=OUT_PCAN.Tx_Dig.In_Dig_33_Sts.MessageEnable  SymbolName=OUT_PCAN_Tx_Dig_In_Dig_33_Sts_MessageEnable_001523  DataType=boolean  Init=0  Slope=1  Bias=0  DataSize=1  fpDataType=boolean  BlockIOType=Outport  DeviceType=0
  out_OUT_PCAN.Tx_Dig.In_Dig_34_Sts.IN_DIG_DIAG : KIBES_Signal/KIBES_Signal  MBDS_LibraryBlock=on  DatabaseKey=1467  SignalName=OUT_PCAN.Tx_Dig.In_Dig_34_Sts.IN_DIG_DIAG  SymbolName=OUT_PCAN_Tx_Dig_In_Dig_34_Sts_IN_DIG_DIAG_001467  DataType=uint16  Init=0  Slope=1  Bias=0  DataSize=1  fpDataType=uint16  BlockIOType=Outport  DeviceType=0
  out_OUT_PCAN.Tx_Dig.In_Dig_34_Sts.IN_DIG_Val : KIBES_Signal/KIBES_Signal  MBDS_LibraryBlock=on  DatabaseKey=1468  SignalName=OUT_PCAN.Tx_Dig.In_Dig_34_Sts.IN_DIG_Val  SymbolName=OUT_PCAN_Tx_Dig_In_Dig_34_Sts_IN_DIG_Val_001468  DataType=boolean  Init=0  Slope=1  Bias=0  DataSize=1  fpDataType=boolean  BlockIOType=Outport  DeviceType=0
  out_OUT_PCAN.Tx_Dig.In_Dig_34_Sts.MessageEnable : KIBES_Signal/KIBES_Signal  MBDS_LibraryBlock=on  DatabaseKey=1524  SignalName=OUT_PCAN.Tx_Dig.In_Dig_34_Sts.MessageEnable  SymbolName=OUT_PCAN_Tx_Dig_In_Dig_34_Sts_MessageEnable_001524  DataType=boolean  Init=0  Slope=1  Bias=0  DataSize=1  fpDataType=boolean  BlockIOType=Outport  DeviceType=0
  out_OUT_PCAN.Tx_Dig.In_Dig_35_Sts.IN_DIG_DIAG : KIBES_Signal/KIBES_Signal  MBDS_LibraryBlock=on  DatabaseKey=1469  SignalName=OUT_PCAN.Tx_Dig.In_Dig_35_Sts.IN_DIG_DIAG  SymbolName=OUT_PCAN_Tx_Dig_In_Dig_35_Sts_IN_DIG_DIAG_001469  DataType=uint16  Init=0  Slope=1  Bias=0  DataSize=1  fpDataType=uint16  BlockIOType=Outport  DeviceType=0
  out_OUT_PCAN.Tx_Dig.In_Dig_35_Sts.IN_DIG_Val : KIBES_Signal/KIBES_Signal  MBDS_LibraryBlock=on  DatabaseKey=1470  SignalName=OUT_PCAN.Tx_Dig.In_Dig_35_Sts.IN_DIG_Val  SymbolName=OUT_PCAN_Tx_Dig_In_Dig_35_Sts_IN_DIG_Val_001470  DataType=boolean  Init=0  Slope=1  Bias=0  DataSize=1  fpDataType=boolean  BlockIOType=Outport  DeviceType=0
  out_OUT_PCAN.Tx_Dig.In_Dig_35_Sts.MessageEnable : KIBES_Signal/KIBES_Signal  MBDS_LibraryBlock=on  DatabaseKey=1525  SignalName=OUT_PCAN.Tx_Dig.In_Dig_35_Sts.MessageEnable  SymbolName=OUT_PCAN_Tx_Dig_In_Dig_35_Sts_MessageEnable_001525  DataType=boolean  Init=0  Slope=1  Bias=0  DataSize=1  fpDataType=boolean  BlockIOType=Outport  DeviceType=0
  out_OUT_PCAN.Tx_Dig.In_Dig_36_Sts.IN_DIG_DIAG : KIBES_Signal/KIBES_Signal  MBDS_LibraryBlock=on  DatabaseKey=1471  SignalName=OUT_PCAN.Tx_Dig.In_Dig_36_Sts.IN_DIG_DIAG  SymbolName=OUT_PCAN_Tx_Dig_In_Dig_36_Sts_IN_DIG_DIAG_001471  DataType=uint16  Init=0  Slope=1  Bias=0  DataSize=1  fpDataType=uint16  BlockIOType=Outport  DeviceType=0
  out_OUT_PCAN.Tx_Dig.In_Dig_36_Sts.IN_DIG_Val : KIBES_Signal/KIBES_Signal  MBDS_LibraryBlock=on  DatabaseKey=1472  SignalName=OUT_PCAN.Tx_Dig.In_Dig_36_Sts.IN_DIG_Val  SymbolName=OUT_PCAN_Tx_Dig_In_Dig_36_Sts_IN_DIG_Val_001472  DataType=boolean  Init=0  Slope=1  Bias=0  DataSize=1  fpDataType=boolean  BlockIOType=Outport  DeviceType=0
  out_OUT_PCAN.Tx_Dig.In_Dig_36_Sts.MessageEnable : KIBES_Signal/KIBES_Signal  MBDS_LibraryBlock=on  DatabaseKey=1526  SignalName=OUT_PCAN.Tx_Dig.In_Dig_36_Sts.MessageEnable  SymbolName=OUT_PCAN_Tx_Dig_In_Dig_36_Sts_MessageEnable_001526  DataType=boolean  Init=0  Slope=1  Bias=0  DataSize=1  fpDataType=boolean  BlockIOType=Outport  DeviceType=0
  out_OUT_PCAN.Tx_Dig.In_Dig_37_Sts.IN_DIG_DIAG : KIBES_Signal/KIBES_Signal  MBDS_LibraryBlock=on  DatabaseKey=1473  SignalName=OUT_PCAN.Tx_Dig.In_Dig_37_Sts.IN_DIG_DIAG  SymbolName=OUT_PCAN_Tx_Dig_In_Dig_37_Sts_IN_DIG_DIAG_001473  DataType=uint16  Init=0  Slope=1  Bias=0  DataSize=1  fpDataType=uint16  BlockIOType=Outport  DeviceType=0
  out_OUT_PCAN.Tx_Dig.In_Dig_37_Sts.IN_DIG_Val : KIBES_Signal/KIBES_Signal  MBDS_LibraryBlock=on  DatabaseKey=1474  SignalName=OUT_PCAN.Tx_Dig.In_Dig_37_Sts.IN_DIG_Val  SymbolName=OUT_PCAN_Tx_Dig_In_Dig_37_Sts_IN_DIG_Val_001474  DataType=boolean  Init=0  Slope=1  Bias=0  DataSize=1  fpDataType=boolean  BlockIOType=Outport  DeviceType=0
  out_OUT_PCAN.Tx_Dig.In_Dig_37_Sts.MessageEnable : KIBES_Signal/KIBES_Signal  MBDS_LibraryBlock=on  DatabaseKey=1527  SignalName=OUT_PCAN.Tx_Dig.In_Dig_37_Sts.MessageEnable  SymbolName=OUT_PCAN_Tx_Dig_In_Dig_37_Sts_MessageEnable_001527  DataType=boolean  Init=0  Slope=1  Bias=0  DataSize=1  fpDataType=boolean  BlockIOType=Outport  DeviceType=0
  out_OUT_PCAN.Tx_Dig.In_Dig_38_Sts.IN_DIG_DIAG : KIBES_Signal/KIBES_Signal  MBDS_LibraryBlock=on  DatabaseKey=1475  SignalName=OUT_PCAN.Tx_Dig.In_Dig_38_Sts.IN_DIG_DIAG  SymbolName=OUT_PCAN_Tx_Dig_In_Dig_38_Sts_IN_DIG_DIAG_001475  DataType=uint16  Init=0  Slope=1  Bias=0  DataSize=1  fpDataType=uint16  BlockIOType=Outport  DeviceType=0
  out_OUT_PCAN.Tx_Dig.In_Dig_38_Sts.IN_DIG_Val : KIBES_Signal/KIBES_Signal  MBDS_LibraryBlock=on  DatabaseKey=1476  SignalName=OUT_PCAN.Tx_Dig.In_Dig_38_Sts.IN_DIG_Val  SymbolName=OUT_PCAN_Tx_Dig_In_Dig_38_Sts_IN_DIG_Val_001476  DataType=boolean  Init=0  Slope=1  Bias=0  DataSize=1  fpDataType=boolean  BlockIOType=Outport  DeviceType=0
  out_OUT_PCAN.Tx_Dig.In_Dig_38_Sts.MessageEnable : KIBES_Signal/KIBES_Signal  MBDS_LibraryBlock=on  DatabaseKey=1528  SignalName=OUT_PCAN.Tx_Dig.In_Dig_38_Sts.MessageEnable  SymbolName=OUT_PCAN_Tx_Dig_In_Dig_38_Sts_MessageEnable_001528  DataType=boolean  Init=0  Slope=1  Bias=0  DataSize=1  fpDataType=boolean  BlockIOType=Outport  DeviceType=0
  out_OUT_PCAN.Tx_Dig.In_Dig_39_Sts.IN_DIG_DIAG : KIBES_Signal/KIBES_Signal  MBDS_LibraryBlock=on  DatabaseKey=1477  SignalName=OUT_PCAN.Tx_Dig.In_Dig_39_Sts.IN_DIG_DIAG  SymbolName=OUT_PCAN_Tx_Dig_In_Dig_39_Sts_IN_DIG_DIAG_001477  DataType=uint16  Init=0  Slope=1  Bias=0  DataSize=1  fpDataType=uint16  BlockIOType=Outport  DeviceType=0
  out_OUT_PCAN.Tx_Dig.In_Dig_39_Sts.IN_DIG_Val : KIBES_Signal/KIBES_Signal  MBDS_LibraryBlock=on  DatabaseKey=1478  SignalName=OUT_PCAN.Tx_Dig.In_Dig_39_Sts.IN_DIG_Val  SymbolName=OUT_PCAN_Tx_Dig_In_Dig_39_Sts_IN_DIG_Val_001478  DataType=boolean  Init=0  Slope=1  Bias=0  DataSize=1  fpDataType=boolean  BlockIOType=Outport  DeviceType=0
  out_OUT_PCAN.Tx_Dig.In_Dig_39_Sts.MessageEnable : KIBES_Signal/KIBES_Signal  MBDS_LibraryBlock=on  DatabaseKey=1529  SignalName=OUT_PCAN.Tx_Dig.In_Dig_39_Sts.MessageEnable  SymbolName=OUT_PCAN_Tx_Dig_In_Dig_39_Sts_MessageEnable_001529  DataType=boolean  Init=0  Slope=1  Bias=0  DataSize=1  fpDataType=boolean  BlockIOType=Outport  DeviceType=0
  out_OUT_PCAN.Tx_Dig.In_Dig_40_Sts.IN_DIG_DIAG : KIBES_Signal/KIBES_Signal  MBDS_LibraryBlock=on  DatabaseKey=1479  SignalName=OUT_PCAN.Tx_Dig.In_Dig_40_Sts.IN_DIG_DIAG  SymbolName=OUT_PCAN_Tx_Dig_In_Dig_40_Sts_IN_DIG_DIAG_001479  DataType=uint16  Init=0  Slope=1  Bias=0  DataSize=1  fpDataType=uint16  BlockIOType=Outport  DeviceType=0
  out_OUT_PCAN.Tx_Dig.In_Dig_40_Sts.IN_DIG_Val : KIBES_Signal/KIBES_Signal  MBDS_LibraryBlock=on  DatabaseKey=1480  SignalName=OUT_PCAN.Tx_Dig.In_Dig_40_Sts.IN_DIG_Val  SymbolName=OUT_PCAN_Tx_Dig_In_Dig_40_Sts_IN_DIG_Val_001480  DataType=boolean  Init=0  Slope=1  Bias=0  DataSize=1  fpDataType=boolean  BlockIOType=Outport  DeviceType=0
  out_OUT_PCAN.Tx_Dig.In_Dig_40_Sts.MessageEnable : KIBES_Signal/KIBES_Signal  MBDS_LibraryBlock=on  DatabaseKey=1530  SignalName=OUT_PCAN.Tx_Dig.In_Dig_40_Sts.MessageEnable  SymbolName=OUT_PCAN_Tx_Dig_In_Dig_40_Sts_MessageEnable_001530  DataType=boolean  Init=0  Slope=1  Bias=0  DataSize=1  fpDataType=boolean  BlockIOType=Outport  DeviceType=0
  out_OUT_PCAN.Tx_Dig.In_Dig_41_Sts.IN_DIG_DIAG : KIBES_Signal/KIBES_Signal  MBDS_LibraryBlock=on  DatabaseKey=1481  SignalName=OUT_PCAN.Tx_Dig.In_Dig_41_Sts.IN_DIG_DIAG  SymbolName=OUT_PCAN_Tx_Dig_In_Dig_41_Sts_IN_DIG_DIAG_001481  DataType=uint16  Init=0  Slope=1  Bias=0  DataSize=1  fpDataType=uint16  BlockIOType=Outport  DeviceType=0
  out_OUT_PCAN.Tx_Dig.In_Dig_41_Sts.IN_DIG_Val : KIBES_Signal/KIBES_Signal  MBDS_LibraryBlock=on  DatabaseKey=1482  SignalName=OUT_PCAN.Tx_Dig.In_Dig_41_Sts.IN_DIG_Val  SymbolName=OUT_PCAN_Tx_Dig_In_Dig_41_Sts_IN_DIG_Val_001482  DataType=boolean  Init=0  Slope=1  Bias=0  DataSize=1  fpDataType=boolean  BlockIOType=Outport  DeviceType=0
  out_OUT_PCAN.Tx_Dig.In_Dig_41_Sts.MessageEnable : KIBES_Signal/KIBES_Signal  MBDS_LibraryBlock=on  DatabaseKey=1531  SignalName=OUT_PCAN.Tx_Dig.In_Dig_41_Sts.MessageEnable  SymbolName=OUT_PCAN_Tx_Dig_In_Dig_41_Sts_MessageEnable_001531  DataType=boolean  Init=0  Slope=1  Bias=0  DataSize=1  fpDataType=boolean  BlockIOType=Outport  DeviceType=0
  out_OUT_PCAN.Tx_Dig.In_Dig_42_Sts.IN_DIG_DIAG : KIBES_Signal/KIBES_Signal  MBDS_LibraryBlock=on  DatabaseKey=1483  SignalName=OUT_PCAN.Tx_Dig.In_Dig_42_Sts.IN_DIG_DIAG  SymbolName=OUT_PCAN_Tx_Dig_In_Dig_42_Sts_IN_DIG_DIAG_001483  DataType=uint16  Init=0  Slope=1  Bias=0  DataSize=1  fpDataType=uint16  BlockIOType=Outport  DeviceType=0
  out_OUT_PCAN.Tx_Dig.In_Dig_42_Sts.IN_DIG_Val : KIBES_Signal/KIBES_Signal  MBDS_LibraryBlock=on  DatabaseKey=1484  SignalName=OUT_PCAN.Tx_Dig.In_Dig_42_Sts.IN_DIG_Val  SymbolName=OUT_PCAN_Tx_Dig_In_Dig_42_Sts_IN_DIG_Val_001484  DataType=boolean  Init=0  Slope=1  Bias=0  DataSize=1  fpDataType=boolean  BlockIOType=Outport  DeviceType=0
  out_OUT_PCAN.Tx_Dig.In_Dig_42_Sts.MessageEnable : KIBES_Signal/KIBES_Signal  MBDS_LibraryBlock=on  DatabaseKey=1532  SignalName=OUT_PCAN.Tx_Dig.In_Dig_42_Sts.MessageEnable  SymbolName=OUT_PCAN_Tx_Dig_In_Dig_42_Sts_MessageEnable_001532  DataType=boolean  Init=0  Slope=1  Bias=0  DataSize=1  fpDataType=boolean  BlockIOType=Outport  DeviceType=0
  out_OUT_PCAN.Tx_Dig.In_Dig_43_Sts.IN_DIG_DIAG : KIBES_Signal/KIBES_Signal  MBDS_LibraryBlock=on  DatabaseKey=1485  SignalName=OUT_PCAN.Tx_Dig.In_Dig_43_Sts.IN_DIG_DIAG  SymbolName=OUT_PCAN_Tx_Dig_In_Dig_43_Sts_IN_DIG_DIAG_001485  DataType=uint16  Init=0  Slope=1  Bias=0  DataSize=1  fpDataType=uint16  BlockIOType=Outport  DeviceType=0
  out_OUT_PCAN.Tx_Dig.In_Dig_43_Sts.IN_DIG_Val : KIBES_Signal/KIBES_Signal  MBDS_LibraryBlock=on  DatabaseKey=1486  SignalName=OUT_PCAN.Tx_Dig.In_Dig_43_Sts.IN_DIG_Val  SymbolName=OUT_PCAN_Tx_Dig_In_Dig_43_Sts_IN_DIG_Val_001486  DataType=boolean  Init=0  Slope=1  Bias=0  DataSize=1  fpDataType=boolean  BlockIOType=Outport  DeviceType=0
  out_OUT_PCAN.Tx_Dig.In_Dig_43_Sts.MessageEnable : KIBES_Signal/KIBES_Signal  MBDS_LibraryBlock=on  DatabaseKey=1533  SignalName=OUT_PCAN.Tx_Dig.In_Dig_43_Sts.MessageEnable  SymbolName=OUT_PCAN_Tx_Dig_In_Dig_43_Sts_MessageEnable_001533  DataType=boolean  Init=0  Slope=1  Bias=0  DataSize=1  fpDataType=boolean  BlockIOType=Outport  DeviceType=0
  out_OUT_PCAN.Tx_Dig.In_Dig_44_Sts.IN_DIG_DIAG : KIBES_Signal/KIBES_Signal  MBDS_LibraryBlock=on  DatabaseKey=1487  SignalName=OUT_PCAN.Tx_Dig.In_Dig_44_Sts.IN_DIG_DIAG  SymbolName=OUT_PCAN_Tx_Dig_In_Dig_44_Sts_IN_DIG_DIAG_001487  DataType=uint16  Init=0  Slope=1  Bias=0  DataSize=1  fpDataType=uint16  BlockIOType=Outport  DeviceType=0
  out_OUT_PCAN.Tx_Dig.In_Dig_44_Sts.IN_DIG_Val : KIBES_Signal/KIBES_Signal  MBDS_LibraryBlock=on  DatabaseKey=1488  SignalName=OUT_PCAN.Tx_Dig.In_Dig_44_Sts.IN_DIG_Val  SymbolName=OUT_PCAN_Tx_Dig_In_Dig_44_Sts_IN_DIG_Val_001488  DataType=boolean  Init=0  Slope=1  Bias=0  DataSize=1  fpDataType=boolean  BlockIOType=Outport  DeviceType=0
  out_OUT_PCAN.Tx_Dig.In_Dig_44_Sts.MessageEnable : KIBES_Signal/KIBES_Signal  MBDS_LibraryBlock=on  DatabaseKey=1534  SignalName=OUT_PCAN.Tx_Dig.In_Dig_44_Sts.MessageEnable  SymbolName=OUT_PCAN_Tx_Dig_In_Dig_44_Sts_MessageEnable_001534  DataType=boolean  Init=0  Slope=1  Bias=0  DataSize=1  fpDataType=boolean  BlockIOType=Outport  DeviceType=0
  out_OUT_PCAN.Tx_Dig.In_Dig_45_Sts.IN_DIG_DIAG : KIBES_Signal/KIBES_Signal  MBDS_LibraryBlock=on  DatabaseKey=1489  SignalName=OUT_PCAN.Tx_Dig.In_Dig_45_Sts.IN_DIG_DIAG  SymbolName=OUT_PCAN_Tx_Dig_In_Dig_45_Sts_IN_DIG_DIAG_001489  DataType=uint16  Init=0  Slope=1  Bias=0  DataSize=1  fpDataType=uint16  BlockIOType=Outport  DeviceType=0
  out_OUT_PCAN.Tx_Dig.In_Dig_45_Sts.IN_DIG_Val : KIBES_Signal/KIBES_Signal  MBDS_LibraryBlock=on  DatabaseKey=1490  SignalName=OUT_PCAN.Tx_Dig.In_Dig_45_Sts.IN_DIG_Val  SymbolName=OUT_PCAN_Tx_Dig_In_Dig_45_Sts_IN_DIG_Val_001490  DataType=boolean  Init=0  Slope=1  Bias=0  DataSize=1  fpDataType=boolean  BlockIOType=Outport  DeviceType=0
  out_OUT_PCAN.Tx_Dig.In_Dig_45_Sts.MessageEnable : KIBES_Signal/KIBES_Signal  MBDS_LibraryBlock=on  DatabaseKey=1535  SignalName=OUT_PCAN.Tx_Dig.In_Dig_45_Sts.MessageEnable  SymbolName=OUT_PCAN_Tx_Dig_In_Dig_45_Sts_MessageEnable_001535  DataType=boolean  Init=0  Slope=1  Bias=0  DataSize=1  fpDataType=boolean  BlockIOType=Outport  DeviceType=0
  out_OUT_PCAN.Tx_Dig.In_Dig_46_Sts.IN_DIG_DIAG : KIBES_Signal/KIBES_Signal  MBDS_LibraryBlock=on  DatabaseKey=1491  SignalName=OUT_PCAN.Tx_Dig.In_Dig_46_Sts.IN_DIG_DIAG  SymbolName=OUT_PCAN_Tx_Dig_In_Dig_46_Sts_IN_DIG_DIAG_001491  DataType=uint16  Init=0  Slope=1  Bias=0  DataSize=1  fpDataType=uint16  BlockIOType=Outport  DeviceType=0
  out_OUT_PCAN.Tx_Dig.In_Dig_46_Sts.IN_DIG_Val : KIBES_Signal/KIBES_Signal  MBDS_LibraryBlock=on  DatabaseKey=1492  SignalName=OUT_PCAN.Tx_Dig.In_Dig_46_Sts.IN_DIG_Val  SymbolName=OUT_PCAN_Tx_Dig_In_Dig_46_Sts_IN_DIG_Val_001492  DataType=boolean  Init=0  Slope=1  Bias=0  DataSize=1  fpDataType=boolean  BlockIOType=Outport  DeviceType=0
  out_OUT_PCAN.Tx_Dig.In_Dig_46_Sts.MessageEnable : KIBES_Signal/KIBES_Signal  MBDS_LibraryBlock=on  DatabaseKey=1536  SignalName=OUT_PCAN.Tx_Dig.In_Dig_46_Sts.MessageEnable  SymbolName=OUT_PCAN_Tx_Dig_In_Dig_46_Sts_MessageEnable_001536  DataType=boolean  Init=0  Slope=1  Bias=0  DataSize=1  fpDataType=boolean  BlockIOType=Outport  DeviceType=0
  out_OUT_PCAN.Tx_Dig.In_Dig_48_Sts.IN_DIG_DIAG : KIBES_Signal/KIBES_Signal  MBDS_LibraryBlock=on  DatabaseKey=1493  SignalName=OUT_PCAN.Tx_Dig.In_Dig_48_Sts.IN_DIG_DIAG  SymbolName=OUT_PCAN_Tx_Dig_In_Dig_48_Sts_IN_DIG_DIAG_001493  DataType=uint16  Init=0  Slope=1  Bias=0  DataSize=1  fpDataType=uint16  BlockIOType=Outport  DeviceType=0
  out_OUT_PCAN.Tx_Dig.In_Dig_48_Sts.IN_DIG_Val : KIBES_Signal/KIBES_Signal  MBDS_LibraryBlock=on  DatabaseKey=1494  SignalName=OUT_PCAN.Tx_Dig.In_Dig_48_Sts.IN_DIG_Val  SymbolName=OUT_PCAN_Tx_Dig_In_Dig_48_Sts_IN_DIG_Val_001494  DataType=boolean  Init=0  Slope=1  Bias=0  DataSize=1  fpDataType=boolean  BlockIOType=Outport  DeviceType=0
  out_OUT_PCAN.Tx_Dig.In_Dig_48_Sts.MessageEnable : KIBES_Signal/KIBES_Signal  MBDS_LibraryBlock=on  DatabaseKey=1537  SignalName=OUT_PCAN.Tx_Dig.In_Dig_48_Sts.MessageEnable  SymbolName=OUT_PCAN_Tx_Dig_In_Dig_48_Sts_MessageEnable_001537  DataType=boolean  Init=0  Slope=1  Bias=0  DataSize=1  fpDataType=boolean  BlockIOType=Outport  DeviceType=0
  out_OUT_PCAN.Tx_Dig.In_Dig_49_Sts.IN_DIG_DIAG : KIBES_Signal/KIBES_Signal  MBDS_LibraryBlock=on  DatabaseKey=1495  SignalName=OUT_PCAN.Tx_Dig.In_Dig_49_Sts.IN_DIG_DIAG  SymbolName=OUT_PCAN_Tx_Dig_In_Dig_49_Sts_IN_DIG_DIAG_001495  DataType=uint16  Init=0  Slope=1  Bias=0  DataSize=1  fpDataType=uint16  BlockIOType=Outport  DeviceType=0
  out_OUT_PCAN.Tx_Dig.In_Dig_49_Sts.IN_DIG_Val : KIBES_Signal/KIBES_Signal  MBDS_LibraryBlock=on  DatabaseKey=1496  SignalName=OUT_PCAN.Tx_Dig.In_Dig_49_Sts.IN_DIG_Val  SymbolName=OUT_PCAN_Tx_Dig_In_Dig_49_Sts_IN_DIG_Val_001496  DataType=boolean  Init=0  Slope=1  Bias=0  DataSize=1  fpDataType=boolean  BlockIOType=Outport  DeviceType=0
  out_OUT_PCAN.Tx_Dig.In_Dig_49_Sts.MessageEnable : KIBES_Signal/KIBES_Signal  MBDS_LibraryBlock=on  DatabaseKey=1538  SignalName=OUT_PCAN.Tx_Dig.In_Dig_49_Sts.MessageEnable  SymbolName=OUT_PCAN_Tx_Dig_In_Dig_49_Sts_MessageEnable_001538  DataType=boolean  Init=0  Slope=1  Bias=0  DataSize=1  fpDataType=boolean  BlockIOType=Outport  DeviceType=0
  out_OUT_PCAN.Tx_Dig.In_Dig_50_Sts.IN_DIG_DIAG : KIBES_Signal/KIBES_Signal  MBDS_LibraryBlock=on  DatabaseKey=1497  SignalName=OUT_PCAN.Tx_Dig.In_Dig_50_Sts.IN_DIG_DIAG  SymbolName=OUT_PCAN_Tx_Dig_In_Dig_50_Sts_IN_DIG_DIAG_001497  DataType=uint16  Init=0  Slope=1  Bias=0  DataSize=1  fpDataType=uint16  BlockIOType=Outport  DeviceType=0
  out_OUT_PCAN.Tx_Dig.In_Dig_50_Sts.IN_DIG_Val : KIBES_Signal/KIBES_Signal  MBDS_LibraryBlock=on  DatabaseKey=1498  SignalName=OUT_PCAN.Tx_Dig.In_Dig_50_Sts.IN_DIG_Val  SymbolName=OUT_PCAN_Tx_Dig_In_Dig_50_Sts_IN_DIG_Val_001498  DataType=boolean  Init=0  Slope=1  Bias=0  DataSize=1  fpDataType=boolean  BlockIOType=Outport  DeviceType=0
  out_OUT_PCAN.Tx_Dig.In_Dig_50_Sts.MessageEnable : KIBES_Signal/KIBES_Signal  MBDS_LibraryBlock=on  DatabaseKey=1539  SignalName=OUT_PCAN.Tx_Dig.In_Dig_50_Sts.MessageEnable  SymbolName=OUT_PCAN_Tx_Dig_In_Dig_50_Sts_MessageEnable_001539  DataType=boolean  Init=0  Slope=1  Bias=0  DataSize=1  fpDataType=boolean  BlockIOType=Outport  DeviceType=0
  wires:
  in_IN_DigitalInputs.IN_DIG_22/1 -> out_OUT_PCAN.Tx_Dig.In_Dig_22_Sts.IN_DIG_Val/1
  in_DIAG_DigitalInputs.IN_DIG_41_DIAG/1 -> out_OUT_PCAN.Tx_Dig.In_Dig_41_Sts.IN_DIG_DIAG/1
  in_DIAG_DigitalInputs.IN_DIG_49_DIAG/1 -> out_OUT_PCAN.Tx_Dig.In_Dig_49_Sts.IN_DIG_DIAG/1
  in_IN_DigitalInputs.IN_DIG_25/1 -> out_OUT_PCAN.Tx_Dig.In_Dig_25_Sts.IN_DIG_Val/1
  in_DIAG_DigitalInputs.IN_DIG_39_DIAG/1 -> out_OUT_PCAN.Tx_Dig.In_Dig_39_Sts.IN_DIG_DIAG/1
  in_IN_DigitalInputs.IN_DIG_50/1 -> out_OUT_PCAN.Tx_Dig.In_Dig_50_Sts.IN_DIG_Val/1
  in_DIAG_DigitalInputs.IN_DIG_42_DIAG/1 -> out_OUT_PCAN.Tx_Dig.In_Dig_42_Sts.IN_DIG_DIAG/1
  in_IN_DigitalInputs.IN_DIG_03/1 -> out_OUT_PCAN.Tx_Dig.In_Dig_03_Sts.IN_DIG_Val/1
  in_IN_DigitalInputs.IN_DIG_05/1 -> out_OUT_PCAN.Tx_Dig.In_Dig_05_Sts.IN_DIG_Val/1
  in_DIAG_DigitalInputs.IN_DIG_36_DIAG/1 -> out_OUT_PCAN.Tx_Dig.In_Dig_36_Sts.IN_DIG_DIAG/1
  in_DIAG_DigitalInputs.IN_DIG_27_DIAG/1 -> out_OUT_PCAN.Tx_Dig.In_Dig_27_Sts.IN_DIG_DIAG/1
  in_DIAG_DigitalInputs.IN_DIG_32_DIAG/1 -> out_OUT_PCAN.Tx_Dig.In_Dig_32_Sts.IN_DIG_DIAG/1
  in_DIAG_DigitalInputs.IN_DIG_31_DIAG/1 -> out_OUT_PCAN.Tx_Dig.In_Dig_31_Sts.IN_DIG_DIAG/1
  in_IN_DigitalInputs.IN_DIG_35/1 -> out_OUT_PCAN.Tx_Dig.In_Dig_35_Sts.IN_DIG_Val/1
  in_IN_DigitalInputs.IN_DIG_48/1 -> out_OUT_PCAN.Tx_Dig.In_Dig_48_Sts.IN_DIG_Val/1
  in_DIAG_DigitalInputs.IN_DIG_48_DIAG/1 -> out_OUT_PCAN.Tx_Dig.In_Dig_48_Sts.IN_DIG_DIAG/1
  in_IN_DigitalInputs.IN_DIG_42/1 -> out_OUT_PCAN.Tx_Dig.In_Dig_42_Sts.IN_DIG_Val/1
  in_IN_DigitalInputs.IN_DIG_49/1 -> out_OUT_PCAN.Tx_Dig.In_Dig_49_Sts.IN_DIG_Val/1
  in_IN_DigitalInputs.IN_DIG_13/1 -> out_OUT_PCAN.Tx_Dig.In_Dig_13_Sts.IN_DIG_Val/1
  in_IN_DigitalInputs.IN_DIG_46/1 -> out_OUT_PCAN.Tx_Dig.In_Dig_46_Sts.IN_DIG_Val/1
  in_IN_DigitalInputs.IN_DIG_12/1 -> out_OUT_PCAN.Tx_Dig.In_Dig_12_Sts.IN_DIG_Val/1
  in_DIAG_DigitalInputs.IN_DIG_44_DIAG/1 -> out_OUT_PCAN.Tx_Dig.In_Dig_44_Sts.IN_DIG_DIAG/1
  in_IN_DigitalInputs.IN_DIG_24/1 -> out_OUT_PCAN.Tx_Dig.In_Dig_24_Sts.IN_DIG_Val/1
  in_IN_DigitalInputs.IN_DIG_45/1 -> out_OUT_PCAN.Tx_Dig.In_Dig_45_Sts.IN_DIG_Val/1
  in_IN_DigitalInputs.IN_DIG_27/1 -> out_OUT_PCAN.Tx_Dig.In_Dig_27_Sts.IN_DIG_Val/1
  in_IN_DigitalInputs.IN_DIG_23/1 -> out_OUT_PCAN.Tx_Dig.In_Dig_23_Sts.IN_DIG_Val/1
  in_DIAG_DigitalInputs.IN_DIG_46_DIAG/1 -> out_OUT_PCAN.Tx_Dig.In_Dig_46_Sts.IN_DIG_DIAG/1
  in_DIAG_DigitalInputs.IN_DIG_43_DIAG/1 -> out_OUT_PCAN.Tx_Dig.In_Dig_43_Sts.IN_DIG_DIAG/1
  in_DIAG_DigitalInputs.IN_DIG_35_DIAG/1 -> out_OUT_PCAN.Tx_Dig.In_Dig_35_Sts.IN_DIG_DIAG/1
  in_DIAG_DigitalInputs.IN_DIG_38_DIAG/1 -> out_OUT_PCAN.Tx_Dig.In_Dig_38_Sts.IN_DIG_DIAG/1
  in_DIAG_DigitalInputs.IN_DIG_34_DIAG/1 -> out_OUT_PCAN.Tx_Dig.In_Dig_34_Sts.IN_DIG_DIAG/1
  in_IN_DigitalInputs.IN_DIG_01/1 -> out_OUT_PCAN.Tx_Dig.In_Dig_01_Sts.IN_DIG_Val/1
  in_IN_DigitalInputs.IN_DIG_32/1 -> out_OUT_PCAN.Tx_Dig.In_Dig_32_Sts.IN_DIG_Val/1
  in_IN_DigitalInputs.IN_DIG_06/1 -> out_OUT_PCAN.Tx_Dig.In_Dig_06_Sts.IN_DIG_Val/1
  in_IN_DigitalInputs.IN_DIG_31/1 -> out_OUT_PCAN.Tx_Dig.In_Dig_31_Sts.IN_DIG_Val/1
  in_DIAG_DigitalInputs.IN_DIG_18_DIAG/1 -> out_OUT_PCAN.Tx_Dig.In_Dig_18_Sts.IN_DIG_DIAG/1
  in_DIAG_DigitalInputs.IN_DIG_07_DIAG/1 -> out_OUT_PCAN.Tx_Dig.In_Dig_07_Sts.IN_DIG_DIAG/1
  in_DIAG_DigitalInputs.IN_DIG_28_DIAG/1 -> out_OUT_PCAN.Tx_Dig.In_Dig_28_Sts.IN_DIG_DIAG/1
  in_IN_DigitalInputs.IN_DIG_28/1 -> out_OUT_PCAN.Tx_Dig.In_Dig_28_Sts.IN_DIG_Val/1
  in_IN_DigitalInputs.IN_DIG_07/1 -> out_OUT_PCAN.Tx_Dig.In_Dig_07_Sts.IN_DIG_Val/1
  in_IN_DigitalInputs.IN_DIG_17/1 -> out_OUT_PCAN.Tx_Dig.In_Dig_17_Sts.IN_DIG_Val/1
  in_DIAG_DigitalInputs.IN_DIG_10_DIAG/1 -> out_OUT_PCAN.Tx_Dig.In_Dig_10_Sts.IN_DIG_DIAG/1
  in_IN_DigitalInputs.IN_DIG_18/1 -> out_OUT_PCAN.Tx_Dig.In_Dig_18_Sts.IN_DIG_Val/1
  in_DIAG_DigitalInputs.IN_DIG_16_DIAG/1 -> out_OUT_PCAN.Tx_Dig.In_Dig_16_Sts.IN_DIG_DIAG/1
  in_IN_DigitalInputs.IN_DIG_21/1 -> out_OUT_PCAN.Tx_Dig.In_Dig_21_Sts.IN_DIG_Val/1
  in_DIAG_DigitalInputs.IN_DIG_45_DIAG/1 -> out_OUT_PCAN.Tx_Dig.In_Dig_45_Sts.IN_DIG_DIAG/1
  in_DIAG_DigitalInputs.IN_DIG_37_DIAG/1 -> out_OUT_PCAN.Tx_Dig.In_Dig_37_Sts.IN_DIG_DIAG/1
  in_DIAG_DigitalInputs.IN_DIG_29_DIAG/1 -> out_OUT_PCAN.Tx_Dig.In_Dig_29_Sts.IN_DIG_DIAG/1
  in_DIAG_DigitalInputs.IN_DIG_11_DIAG/1 -> out_OUT_PCAN.Tx_Dig.In_Dig_11_Sts.IN_DIG_DIAG/1
  in_IN_DigitalInputs.IN_DIG_16/1 -> out_OUT_PCAN.Tx_Dig.In_Dig_16_Sts.IN_DIG_Val/1
  in_DIAG_DigitalInputs.IN_DIG_04_DIAG/1 -> out_OUT_PCAN.Tx_Dig.In_Dig_04_Sts.IN_DIG_DIAG/1
  in_IN_DigitalInputs.IN_DIG_26/1 -> out_OUT_PCAN.Tx_Dig.In_Dig_26_Sts.IN_DIG_Val/1
  in_DIAG_DigitalInputs.IN_DIG_09_DIAG/1 -> out_OUT_PCAN.Tx_Dig.In_Dig_09_Sts.IN_DIG_DIAG/1
  in_IN_DigitalInputs.IN_DIG_09/1 -> out_OUT_PCAN.Tx_Dig.In_Dig_09_Sts.IN_DIG_Val/1
  in_IN_DigitalInputs.IN_DIG_08/1 -> out_OUT_PCAN.Tx_Dig.In_Dig_08_Sts.IN_DIG_Val/1
  in_IN_DigitalInputs.IN_DIG_02/1 -> out_OUT_PCAN.Tx_Dig.In_Dig_02_Sts.IN_DIG_Val/1
  in_IN_DigitalInputs.IN_DIG_36/1 -> out_OUT_PCAN.Tx_Dig.In_Dig_36_Sts.IN_DIG_Val/1
  in_DIAG_DigitalInputs.IN_DIG_15_DIAG/1 -> out_OUT_PCAN.Tx_Dig.In_Dig_15_Sts.IN_DIG_DIAG/1
  in_DIAG_DigitalInputs.IN_DIG_06_DIAG/1 -> out_OUT_PCAN.Tx_Dig.In_Dig_06_Sts.IN_DIG_DIAG/1
  in_IN_DigitalInputs.IN_DIG_38/1 -> out_OUT_PCAN.Tx_Dig.In_Dig_38_Sts.IN_DIG_Val/1
  in_IN_DigitalInputs.IN_DIG_29/1 -> out_OUT_PCAN.Tx_Dig.In_Dig_29_Sts.IN_DIG_Val/1
  in_DIAG_DigitalInputs.IN_DIG_14_DIAG/1 -> out_OUT_PCAN.Tx_Dig.In_Dig_14_Sts.IN_DIG_DIAG/1
  in_IN_DigitalInputs.IN_DIG_14/1 -> out_OUT_PCAN.Tx_Dig.In_Dig_14_Sts.IN_DIG_Val/1
  in_IN_DigitalInputs.IN_DIG_33/1 -> out_OUT_PCAN.Tx_Dig.In_Dig_33_Sts.IN_DIG_Val/1
  in_IN_DigitalInputs.IN_DIG_19/1 -> out_OUT_PCAN.Tx_Dig.In_Dig_19_Sts.IN_DIG_Val/1
  in_DIAG_DigitalInputs.IN_DIG_13_DIAG/1 -> out_OUT_PCAN.Tx_Dig.In_Dig_13_Sts.IN_DIG_DIAG/1
  in_DIAG_DigitalInputs.IN_DIG_12_DIAG/1 -> out_OUT_PCAN.Tx_Dig.In_Dig_12_Sts.IN_DIG_DIAG/1
  in_DIAG_DigitalInputs.IN_DIG_21_DIAG/1 -> out_OUT_PCAN.Tx_Dig.In_Dig_21_Sts.IN_DIG_DIAG/1
  in_IN_DigitalInputs.IN_DIG_10/1 -> out_OUT_PCAN.Tx_Dig.In_Dig_10_Sts.IN_DIG_Val/1
  in_DIAG_DigitalInputs.IN_DIG_22_DIAG/1 -> out_OUT_PCAN.Tx_Dig.In_Dig_22_Sts.IN_DIG_DIAG/1
  in_IN_DigitalInputs.IN_DIG_11/1 -> out_OUT_PCAN.Tx_Dig.In_Dig_11_Sts.IN_DIG_Val/1
  in_DIAG_DigitalInputs.IN_DIG_23_DIAG/1 -> out_OUT_PCAN.Tx_Dig.In_Dig_23_Sts.IN_DIG_DIAG/1
  in_DIAG_DigitalInputs.IN_DIG_03_DIAG/1 -> out_OUT_PCAN.Tx_Dig.In_Dig_03_Sts.IN_DIG_DIAG/1
  in_IN_DigitalInputs.IN_DIG_40/1 -> out_OUT_PCAN.Tx_Dig.In_Dig_40_Sts.IN_DIG_Val/1
  in_IN_DigitalInputs.IN_DIG_43/1 -> out_OUT_PCAN.Tx_Dig.In_Dig_43_Sts.IN_DIG_Val/1
  in_DIAG_DigitalInputs.IN_DIG_33_DIAG/1 -> out_OUT_PCAN.Tx_Dig.In_Dig_33_Sts.IN_DIG_DIAG/1
  in_IN_DigitalInputs.IN_DIG_44/1 -> out_OUT_PCAN.Tx_Dig.In_Dig_44_Sts.IN_DIG_Val/1
  in_IN_DigitalInputs.IN_DIG_15/1 -> out_OUT_PCAN.Tx_Dig.In_Dig_15_Sts.IN_DIG_Val/1
  in_DIAG_DigitalInputs.IN_DIG_20_DIAG/1 -> out_OUT_PCAN.Tx_Dig.In_Dig_20_Sts.IN_DIG_DIAG/1
  in_DIAG_DigitalInputs.IN_DIG_17_DIAG/1 -> out_OUT_PCAN.Tx_Dig.In_Dig_17_Sts.IN_DIG_DIAG/1
  in_IN_DigitalInputs.IN_DIG_20/1 -> out_OUT_PCAN.Tx_Dig.In_Dig_20_Sts.IN_DIG_Val/1
  in_DIAG_DigitalInputs.IN_DIG_30_DIAG/1 -> out_OUT_PCAN.Tx_Dig.In_Dig_30_Sts.IN_DIG_DIAG/1
  in_DIAG_DigitalInputs.IN_DIG_50_DIAG/1 -> out_OUT_PCAN.Tx_Dig.In_Dig_50_Sts.IN_DIG_DIAG/1
  in_DIAG_DigitalInputs.IN_DIG_05_DIAG/1 -> out_OUT_PCAN.Tx_Dig.In_Dig_05_Sts.IN_DIG_DIAG/1
  in_DIAG_DigitalInputs.IN_DIG_02_DIAG/1 -> out_OUT_PCAN.Tx_Dig.In_Dig_02_Sts.IN_DIG_DIAG/1
  in_DIAG_DigitalInputs.IN_DIG_25_DIAG/1 -> out_OUT_PCAN.Tx_Dig.In_Dig_25_Sts.IN_DIG_DIAG/1
  bo_SendEnable/1 -> out_OUT_PCAN.Tx_Dig.In_Dig_49_Sts.MessageEnable/1, out_OUT_PCAN.Tx_Dig.In_Dig_50_Sts.MessageEnable/1, out_OUT_PCAN.Tx_Dig.In_Dig_48_Sts.MessageEnable/1, out_OUT_PCAN.Tx_Dig.In_Dig_46_Sts.MessageEnable/1, out_OUT_PCAN.Tx_Dig.In_Dig_45_Sts.MessageEnable/1, out_OUT_PCAN.Tx_Dig.In_Dig_44_Sts.MessageEnable/1, out_OUT_PCAN.Tx_Dig.In_Dig_43_Sts.MessageEnable/1, out_OUT_PCAN.Tx_Dig.In_Dig_42_Sts.MessageEnable/1, out_OUT_PCAN.Tx_Dig.In_Dig_41_Sts.MessageEnable/1, out_OUT_PCAN.Tx_Dig.In_Dig_40_Sts.MessageEnable/1, out_OUT_PCAN.Tx_Dig.In_Dig_39_Sts.MessageEnable/1, out_OUT_PCAN.Tx_Dig.In_Dig_38_Sts.MessageEnable/1, out_OUT_PCAN.Tx_Dig.In_Dig_37_Sts.MessageEnable/1, out_OUT_PCAN.Tx_Dig.In_Dig_36_Sts.MessageEnable/1, out_OUT_PCAN.Tx_Dig.In_Dig_35_Sts.MessageEnable/1, out_OUT_PCAN.Tx_Dig.In_Dig_34_Sts.MessageEnable/1, out_OUT_PCAN.Tx_Dig.In_Dig_33_Sts.MessageEnable/1, out_OUT_PCAN.Tx_Dig.In_Dig_32_Sts.MessageEnable/1, out_OUT_PCAN.Tx_Dig.In_Dig_31_Sts.MessageEnable/1, out_OUT_PCAN.Tx_Dig.In_Dig_30_Sts.MessageEnable/1, out_OUT_PCAN.Tx_Dig.In_Dig_29_Sts.MessageEnable/1, out_OUT_PCAN.Tx_Dig.In_Dig_28_Sts.MessageEnable/1, out_OUT_PCAN.Tx_Dig.In_Dig_27_Sts.MessageEnable/1, out_OUT_PCAN.Tx_Dig.In_Dig_26_Sts.MessageEnable/1, out_OUT_PCAN.Tx_Dig.In_Dig_25_Sts.MessageEnable/1, out_OUT_PCAN.Tx_Dig.In_Dig_24_Sts.MessageEnable/1, out_OUT_PCAN.Tx_Dig.In_Dig_23_Sts.MessageEnable/1, out_OUT_PCAN.Tx_Dig.In_Dig_22_Sts.MessageEnable/1, out_OUT_PCAN.Tx_Dig.In_Dig_21_Sts.MessageEnable/1, out_OUT_PCAN.Tx_Dig.In_Dig_20_Sts.MessageEnable/1, out_OUT_PCAN.Tx_Dig.In_Dig_19_Sts.MessageEnable/1, out_OUT_PCAN.Tx_Dig.In_Dig_18_Sts.MessageEnable/1, out_OUT_PCAN.Tx_Dig.In_Dig_17_Sts.MessageEnable/1, out_OUT_PCAN.Tx_Dig.In_Dig_16_Sts.MessageEnable/1, out_OUT_PCAN.Tx_Dig.In_Dig_15_Sts.MessageEnable/1, out_OUT_PCAN.Tx_Dig.In_Dig_14_Sts.MessageEnable/1, out_OUT_PCAN.Tx_Dig.In_Dig_13_Sts.MessageEnable/1, out_OUT_PCAN.Tx_Dig.In_Dig_12_Sts.MessageEnable/1, out_OUT_PCAN.Tx_Dig.In_Dig_11_Sts.MessageEnable/1, out_OUT_PCAN.Tx_Dig.In_Dig_10_Sts.MessageEnable/1, out_OUT_PCAN.Tx_Dig.In_Dig_09_Sts.MessageEnable/1, out_OUT_PCAN.Tx_Dig.In_Dig_08_Sts.MessageEnable/1, out_OUT_PCAN.Tx_Dig.In_Dig_07_Sts.MessageEnable/1, out_OUT_PCAN.Tx_Dig.In_Dig_06_Sts.MessageEnable/1, out_OUT_PCAN.Tx_Dig.In_Dig_05_Sts.MessageEnable/1, out_OUT_PCAN.Tx_Dig.In_Dig_04_Sts.MessageEnable/1, out_OUT_PCAN.Tx_Dig.In_Dig_03_Sts.MessageEnable/1, out_OUT_PCAN.Tx_Dig.In_Dig_02_Sts.MessageEnable/1, out_OUT_PCAN.Tx_Dig.In_Dig_01_Sts.MessageEnable/1
  in_IN_DigitalInputs.IN_DIG_04/1 -> out_OUT_PCAN.Tx_Dig.In_Dig_04_Sts.IN_DIG_Val/1
  in_DIAG_DigitalInputs.IN_DIG_40_DIAG/1 -> out_OUT_PCAN.Tx_Dig.In_Dig_40_Sts.IN_DIG_DIAG/1
  in_DIAG_DigitalInputs.IN_DIG_19_DIAG/1 -> out_OUT_PCAN.Tx_Dig.In_Dig_19_Sts.IN_DIG_DIAG/1
  in_IN_DigitalInputs.IN_DIG_39/1 -> out_OUT_PCAN.Tx_Dig.In_Dig_39_Sts.IN_DIG_Val/1
  in_IN_DigitalInputs.IN_DIG_34/1 -> out_OUT_PCAN.Tx_Dig.In_Dig_34_Sts.IN_DIG_Val/1
  in_DIAG_DigitalInputs.IN_DIG_08_DIAG/1 -> out_OUT_PCAN.Tx_Dig.In_Dig_08_Sts.IN_DIG_DIAG/1
  in_IN_DigitalInputs.IN_DIG_41/1 -> out_OUT_PCAN.Tx_Dig.In_Dig_41_Sts.IN_DIG_Val/1
  in_DIAG_DigitalInputs.IN_DIG_24_DIAG/1 -> out_OUT_PCAN.Tx_Dig.In_Dig_24_Sts.IN_DIG_DIAG/1
  in_DIAG_DigitalInputs.IN_DIG_26_DIAG/1 -> out_OUT_PCAN.Tx_Dig.In_Dig_26_Sts.IN_DIG_DIAG/1
  in_DIAG_DigitalInputs.IN_DIG_01_DIAG/1 -> out_OUT_PCAN.Tx_Dig.In_Dig_01_Sts.IN_DIG_DIAG/1
  in_IN_DigitalInputs.IN_DIG_30/1 -> out_OUT_PCAN.Tx_Dig.In_Dig_30_Sts.IN_DIG_Val/1
  in_IN_DigitalInputs.IN_DIG_37/1 -> out_OUT_PCAN.Tx_Dig.In_Dig_37_Sts.IN_DIG_Val/1
